simulink model "IEEE123bus_v2019b_Phasor_DPL_ZIPload"  (R2019b)
(part 2 of 12)

  54-55 1 : powerlib/Elements/Distributed Parameters Line  Phases=3  Frequency=60  Resistance=R_1  Inductance=L_1  Capacitance=C_1  Length=275*ft2km  x1=[438.133979265469 4196.77368982038 4204.09231927321;376.991118430775 376.991118430775 376.991118430775;1.68907178229158 -2.40712758914085 2.30524752746821]  x2=[438.133982703911 4196.77368424004 4204.09238504697;376.991118430775 376.991118430775 376.991118430775;1.68907225438477 -2.40712762517757 2.30524750308445]  x3=[0.57767960711374 15.661337452475 12.3899368514742;376.991118430775 376.991118430775 376.991118430775;1.69020592810727 -2.4073134537239 2.30498818329341]  x4=[0.574053544355369 15.6695231741292 12.3933369767456;376.991118430775 376.991118430775 376.991118430775;1.68780051280511 -2.40704970753644 2.30539938237483]  x5=3.44891242524002e-07  V1=ones(3,3)  V2=ones(3,3)  I1=ones(3,3)  I2=ones(3,3)  nHarmo=1  Measurements=None
      settings: SourceProductName=Simscape Electrical
  54-57 3 : powerlib/Elements/Distributed Parameters Line  Phases=3  Frequency=60  Resistance=R_3  Inductance=L_3  Capacitance=C_3  Length=350*ft2km  x1=[442.148345522071 4196.71640972957 4204.09408929467;376.991118430775 376.991118430775 376.991118430775;-0.415145669536993 0.209794158961751 1.78266979920928]  x2=[442.443441248541 4205.29068825861 4210.86387558391;376.991118430775 376.991118430775 376.991118430775;-0.41559689824482 0.208885412947149 1.78176090411138]  x3=[2.56674775762388 185.771024626491 185.574933274428;376.991118430775 376.991118430775 376.991118430775;-1.9761686452555 -1.30181532404798 0.286194361532175]  x4=[2.80709832831061 185.943793008895 185.884239198519;376.991118430775 376.991118430775 376.991118430775;0.738398999629426 1.70643542841195 -3.02471127566214]  x5=4.38952490485094e-07  V1=ones(3,3)  V2=ones(3,3)  I1=ones(3,3)  I2=ones(3,3)  nHarmo=1  Measurements=None
      settings: SourceProductName=Simscape Electrical
  55 : powerlib/Measurements/Three-Phase V-I Measurement  VoltageMeasurement=phase-to-ground  SetLabelV=on  LabelV=V55  Vpu=off  VpuLL=off  CurrentMeasurement=no  SetLabelI=on  LabelI=I65  Ipu=off  Pbase=100e6  Vbase=24900  OutputType=Complex  PhasorSimulation=on  PSBequivalent=0
      settings: SourceProductName=Simscape Electrical
  55 Y Z : Subsystem  mask(Single Phase ZIP Load){Vnom=1.0*2401.78, fnom=60, Pnom=20e3*a, Qnom=10e3*a, LoadType=Constant Z, Vlim=0.7}
      mask prompts: Vnom "Nominal Voltage Vn (Vrms)"; fnom "Nominal Frequency fn (Hz)"; Pnom "Nominal Active power (W)"; Qnom "Nominal Reactive power (VAR)"; LoadType "Load Type"; Vlim "Minimum voltage (pu)"
      mask help:
      | Notes:
      | Single Phase ZIP load model which gets converted to constant Z type if the voltage becomes lower than the Minimum Voltage.
      mask TypeOptions LoadType: Constant Z | constant I | constant P
      mask DialogControl ParameterTabVar0 Prompt: Parameters
      mask DialogControl ParameterTabVar1 Prompt: Type
      mask Display:
      | color('red');
      | A=[-210,-180,-170,-160,-147,-140,-130,-120,-110,-80,-50,-49,-45,-39,-33,-26,-21,-18,-17,-19,-22,-22,-26,-27,-25,-22,-16,-9,-3,2,6,6,4,1,1,-3,-4,-2,2,7,14,20,26,29,30,28,24,24,21,20,21,25,31,37,44,49,50,50,80];
      | B=[-41.5,-41.5,-63,-20,-63,-20,-63,-20,-41.5,-41.5,-41.5,-34,-26,-21,-20,-22,-28,-37,-47,-57,-63,-63,-54,-44,-34,-26,-21,-20,-22,-28,-37,-47,-57,-63,-63,-54,-44,-34,-26,-21,-20,-22,-28,-37,-47,-57,-63,-63,-54,-44,-34,-26,-21,-20,-22,-28,-37,-41.50,-41.5];
      | plot(A,B);
      | color('black');
      | port_label('LConn', 1, '+')
  55-56 1 : powerlib/Elements/Distributed Parameters Line  Phases=3  Frequency=60  Resistance=R_1  Inductance=L_1  Capacitance=C_1  Length=275*ft2km  x1=[438.133982703911 4196.77368424004 4204.09238504697;376.991118430775 376.991118430775 376.991118430775;1.68907225438477 -2.40712762517757 2.30524750308445]  x2=[438.134165148188 4196.77369074888 4204.09236912075;376.991118430775 376.991118430775 376.991118430775;1.68907249725304 -2.4071276498981 2.30524750155646]  x3=[0.577431411639377 15.6627739559426 12.3913283618648;376.991118430775 376.991118430775 376.991118430775;1.68689993805843 -2.40728955810454 2.30521819631482]  x4=[0.574303722649217 15.6680865843111 12.391945096847;376.991118430775 376.991118430775 376.991118430775;1.69112626810043 -2.40707363161943 2.30516940106888]  x5=3.44891242524002e-07  V1=ones(3,3)  V2=ones(3,3)  I1=ones(3,3)  I2=ones(3,3)  nHarmo=1  Measurements=None
      settings: SourceProductName=Simscape Electrical
  56 : powerlib/Measurements/Three-Phase V-I Measurement  VoltageMeasurement=phase-to-ground  SetLabelV=on  LabelV=V56  Vpu=off  VpuLL=off  CurrentMeasurement=no  SetLabelI=on  LabelI=I65  Ipu=off  Pbase=100e6  Vbase=24900  OutputType=Complex  PhasorSimulation=on  PSBequivalent=0
      settings: SourceProductName=Simscape Electrical
  56 Y PQ : Subsystem  mask(Single Phase ZIP Load){Vnom=1.0*2401.78, fnom=60, Pnom=20e3*a, Qnom=10e3*a, LoadType=constant P, Vlim=0.7}
      mask prompts: Vnom "Nominal Voltage Vn (Vrms)"; fnom "Nominal Frequency fn (Hz)"; Pnom "Nominal Active power (W)"; Qnom "Nominal Reactive power (VAR)"; LoadType "Load Type"; Vlim "Minimum voltage (pu)"
      mask help:
      | Notes:
      | Single Phase ZIP load model which gets converted to constant Z type if the voltage becomes lower than the Minimum Voltage.
      mask TypeOptions LoadType: Constant Z | constant I | constant P
      mask DialogControl ParameterTabVar0 Prompt: Parameters
      mask DialogControl ParameterTabVar1 Prompt: Type
      mask Display:
      | color('red');
      | A=[-210,-180,-170,-160,-147,-140,-130,-120,-110,-80,-50,-49,-45,-39,-33,-26,-21,-18,-17,-19,-22,-22,-26,-27,-25,-22,-16,-9,-3,2,6,6,4,1,1,-3,-4,-2,2,7,14,20,26,29,30,28,24,24,21,20,21,25,31,37,44,49,50,50,80];
      | B=[-41.5,-41.5,-63,-20,-63,-20,-63,-20,-41.5,-41.5,-41.5,-34,-26,-21,-20,-22,-28,-37,-47,-57,-63,-63,-54,-44,-34,-26,-21,-20,-22,-28,-37,-47,-57,-63,-63,-54,-44,-34,-26,-21,-20,-22,-28,-37,-47,-57,-63,-63,-54,-44,-34,-26,-21,-20,-22,-28,-37,-41.50,-41.5];
      | plot(A,B);
      | color('black');
      | port_label('LConn', 1, '+')
  57 : powerlib/Measurements/Three-Phase V-I Measurement  VoltageMeasurement=phase-to-ground  SetLabelV=on  LabelV=V57  Vpu=off  VpuLL=off  CurrentMeasurement=no  SetLabelI=on  LabelI=I65  Ipu=off  Pbase=100e6  Vbase=24900  OutputType=Complex  PhasorSimulation=on  PSBequivalent=0
      settings: SourceProductName=Simscape Electrical
  57-58 10 : powerlib/Elements/Distributed Parameters Line  Phases=1  Frequency=60  Resistance=R_10(2,2)  Inductance=L_10(2,2)  Capacitance=C_10(2,2)  Length=250*ft2km  x1=[3435.43252192825;376.991118430775;-2.0999098236995]  x2=[3435.43292902942;376.991118430775;-2.09990968882398]  x3=[6.29780376901278;376.991118430775;-2.09990516681349]  x4=[6.28406360517737;376.991118430775;-2.100031331049]  x5=3.09938851618982e-07  V1=[2.049e+04;377;-2.115]  V2=[2.048e+04;377;-2.115]  I1=[33.62;377;-2.106]  I2=[35.2;377;-2.126]  nHarmo=1  Measurements=None
      settings: SourceProductName=Simscape Electrical
  57-60 3 : powerlib/Elements/Distributed Parameters Line  Phases=3  Frequency=60  Resistance=R_3  Inductance=L_3  Capacitance=C_3  Length=750*ft2km  x1=[442.443441248541 4205.29068825861 4210.86387558391;376.991118430775 376.991118430775 376.991118430775;-0.415786019605193 0.20872918428044 1.78160399294376]  x2=[443.077137686739 4223.67526780051 4225.38226709269;376.991118430775 376.991118430775 376.991118430775;-0.416751865838829 0.206794419050763 1.77966624251521]  x3=[2.57085014444712 185.772514480957 185.583387037946;376.991118430775 376.991118430775 376.991118430775;-1.97623221125093 -1.30182578459823 0.286182634176113]  x4=[2.81031115790824 185.910223378036 185.848218088083;376.991118430775 376.991118430775 376.991118430775;0.738408797497777 1.70599063264223 -3.02515609310221]  x5=9.40612479610915e-07  V1=ones(3,3)  V2=ones(3,3)  I1=ones(3,3)  I2=ones(3,3)  nHarmo=1  Measurements=None
      settings: SourceProductName=Simscape Electrical
  58 : Subsystem
  58 Y I : Subsystem  mask(Single Phase ZIP Load){Vnom=1.0*2401.78, fnom=60, Pnom=20e3*a, Qnom=10e3*a, LoadType=constant I, Vlim=0.7}
      mask prompts: Vnom "Nominal Voltage Vn (Vrms)"; fnom "Nominal Frequency fn (Hz)"; Pnom "Nominal Active power (W)"; Qnom "Nominal Reactive power (VAR)"; LoadType "Load Type"; Vlim "Minimum voltage (pu)"
      mask help:
      | Notes:
      | Single Phase ZIP load model which gets converted to constant Z type if the voltage becomes lower than the Minimum Voltage.
      mask TypeOptions LoadType: Constant Z | constant I | constant P
      mask DialogControl ParameterTabVar0 Prompt: Parameters
      mask DialogControl ParameterTabVar1 Prompt: Type
      mask Display:
      | color('red');
      | A=[-210,-180,-170,-160,-147,-140,-130,-120,-110,-80,-50,-49,-45,-39,-33,-26,-21,-18,-17,-19,-22,-22,-26,-27,-25,-22,-16,-9,-3,2,6,6,4,1,1,-3,-4,-2,2,7,14,20,26,29,30,28,24,24,21,20,21,25,31,37,44,49,50,50,80];
      | B=[-41.5,-41.5,-63,-20,-63,-20,-63,-20,-41.5,-41.5,-41.5,-34,-26,-21,-20,-22,-28,-37,-47,-57,-63,-63,-54,-44,-34,-26,-21,-20,-22,-28,-37,-47,-57,-63,-63,-54,-44,-34,-26,-21,-20,-22,-28,-37,-47,-57,-63,-63,-54,-44,-34,-26,-21,-20,-22,-28,-37,-41.50,-41.5];
      | plot(A,B);
      | color('black');
      | port_label('LConn', 1, '+')
  58-59 10 : powerlib/Elements/Distributed Parameters Line  Phases=1  Frequency=60  Resistance=R_10(2,2)  Inductance=L_10(2,2)  Capacitance=C_10(2,2)  Length=10*ft2km  x1=[3435.43251331732;376.991118430775;-2.09979765583582]  x2=[3435.43252192825;376.991118430775;-2.09979765327296]  x3=[6.29489077198716;376.991118430775;-2.09979765558234]  x4=[6.28801994262156;376.991118430775;-2.09980232984339]  x5=1.23975540647593e-08  V1=[2.049e+04;377;-2.115]  V2=[2.048e+04;377;-2.115]  I1=[33.62;377;-2.106]  I2=[35.2;377;-2.126]  nHarmo=1  Measurements=None
      settings: SourceProductName=Simscape Electrical
  59 : Subsystem
  59 Y PQ : Subsystem  mask(Single Phase ZIP Load){Vnom=1.0*2401.78, fnom=60, Pnom=20e3*a, Qnom=10e3*a, LoadType=constant P, Vlim=0.7}
      mask prompts: Vnom "Nominal Voltage Vn (Vrms)"; fnom "Nominal Frequency fn (Hz)"; Pnom "Nominal Active power (W)"; Qnom "Nominal Reactive power (VAR)"; LoadType "Load Type"; Vlim "Minimum voltage (pu)"
      mask help:
      | Notes:
      | Single Phase ZIP load model which gets converted to constant Z type if the voltage becomes lower than the Minimum Voltage.
      mask TypeOptions LoadType: Constant Z | constant I | constant P
      mask DialogControl ParameterTabVar0 Prompt: Parameters
      mask DialogControl ParameterTabVar1 Prompt: Type
      mask Display:
      | color('red');
      | A=[-210,-180,-170,-160,-147,-140,-130,-120,-110,-80,-50,-49,-45,-39,-33,-26,-21,-18,-17,-19,-22,-22,-26,-27,-25,-22,-16,-9,-3,2,6,6,4,1,1,-3,-4,-2,2,7,14,20,26,29,30,28,24,24,21,20,21,25,31,37,44,49,50,50,80];
      | B=[-41.5,-41.5,-63,-20,-63,-20,-63,-20,-41.5,-41.5,-41.5,-34,-26,-21,-20,-22,-28,-37,-47,-57,-63,-63,-54,-44,-34,-26,-21,-20,-22,-28,-37,-47,-57,-63,-63,-54,-44,-34,-26,-21,-20,-22,-28,-37,-47,-57,-63,-63,-54,-44,-34,-26,-21,-20,-22,-28,-37,-41.50,-41.5];
      | plot(A,B);
      | color('black');
      | port_label('LConn', 1, '+')
  59-94 : powerlib/Elements/Breaker  InitialState=0  SwitchingTimes="[1/60  5/60]"  External=off  BreakerResistance=0.01  SnubberResistance=1e6  SnubberCapacitance=inf  Measurements=None  MoreParameters=on  NoBreakLoop=off
      settings: SourceProductName=Simscape Electrical
  6 : Subsystem
  6 Y Z : Subsystem  mask(Single Phase ZIP Load){Vnom=1.0*2401.78, fnom=60, Pnom=40e3*a, Qnom=20e3*a, LoadType=Constant Z, Vlim=0.7}
      mask prompts: Vnom "Nominal Voltage Vn (Vrms)"; fnom "Nominal Frequency fn (Hz)"; Pnom "Nominal Active power (W)"; Qnom "Nominal Reactive power (VAR)"; LoadType "Load Type"; Vlim "Minimum voltage (pu)"
      mask help:
      | Notes:
      | Single Phase ZIP load model which gets converted to constant Z type if the voltage becomes lower than the Minimum Voltage.
      mask TypeOptions LoadType: Constant Z | constant I | constant P
      mask DialogControl ParameterTabVar0 Prompt: Parameters
      mask DialogControl ParameterTabVar1 Prompt: Type
      mask Display:
      | color('red');
      | A=[-210,-180,-170,-160,-147,-140,-130,-120,-110,-80,-50,-49,-45,-39,-33,-26,-21,-18,-17,-19,-22,-22,-26,-27,-25,-22,-16,-9,-3,2,6,6,4,1,1,-3,-4,-2,2,7,14,20,26,29,30,28,24,24,21,20,21,25,31,37,44,49,50,50,80];
      | B=[-41.5,-41.5,-63,-20,-63,-20,-63,-20,-41.5,-41.5,-41.5,-34,-26,-21,-20,-22,-28,-37,-47,-57,-63,-63,-54,-44,-34,-26,-21,-20,-22,-28,-37,-47,-57,-63,-63,-54,-44,-34,-26,-21,-20,-22,-28,-37,-47,-57,-63,-63,-54,-44,-34,-26,-21,-20,-22,-28,-37,-41.50,-41.5];
      | plot(A,B);
      | color('black');
      | port_label('LConn', 1, '+')
  60 : powerlib/Measurements/Three-Phase V-I Measurement  VoltageMeasurement=phase-to-ground  SetLabelV=on  LabelV=V60  Vpu=off  VpuLL=off  CurrentMeasurement=no  SetLabelI=on  LabelI=I65  Ipu=off  Pbase=100e6  Vbase=24900  OutputType=Complex  PhasorSimulation=on  PSBequivalent=0
      settings: SourceProductName=Simscape Electrical
  60 Y PQ : Subsystem  mask(Single Phase ZIP Load){Vnom=1.0*2401.78, fnom=60, Pnom=20e3*a, Qnom=10e3*a, LoadType=constant P, Vlim=0.7}
      mask prompts: Vnom "Nominal Voltage Vn (Vrms)"; fnom "Nominal Frequency fn (Hz)"; Pnom "Nominal Active power (W)"; Qnom "Nominal Reactive power (VAR)"; LoadType "Load Type"; Vlim "Minimum voltage (pu)"
      mask help:
      | Notes:
      | Single Phase ZIP load model which gets converted to constant Z type if the voltage becomes lower than the Minimum Voltage.
      mask TypeOptions LoadType: Constant Z | constant I | constant P
      mask DialogControl ParameterTabVar0 Prompt: Parameters
      mask DialogControl ParameterTabVar1 Prompt: Type
      mask Display:
      | color('red');
      | A=[-210,-180,-170,-160,-147,-140,-130,-120,-110,-80,-50,-49,-45,-39,-33,-26,-21,-18,-17,-19,-22,-22,-26,-27,-25,-22,-16,-9,-3,2,6,6,4,1,1,-3,-4,-2,2,7,14,20,26,29,30,28,24,24,21,20,21,25,31,37,44,49,50,50,80];
      | B=[-41.5,-41.5,-63,-20,-63,-20,-63,-20,-41.5,-41.5,-41.5,-34,-26,-21,-20,-22,-28,-37,-47,-57,-63,-63,-54,-44,-34,-26,-21,-20,-22,-28,-37,-47,-57,-63,-63,-54,-44,-34,-26,-21,-20,-22,-28,-37,-47,-57,-63,-63,-54,-44,-34,-26,-21,-20,-22,-28,-37,-41.50,-41.5];
      | plot(A,B);
      | color('black');
      | port_label('LConn', 1, '+')
  60-1 : powerlib/Elements/Three-Phase Breaker  InitialState=closed  SwitchA=off  SwitchB=off  SwitchC=off  SwitchTimes="[1/60  5/60]"  External=off  BreakerResistance=1e-6  SnubberResistance=1e6  SnubberCapacitance=inf  Measurements=None
      settings: SourceProductName=Simscape Electrical
  60-61 5 : powerlib/Elements/Distributed Parameters Line  Phases=3  Frequency=60  Resistance=R_5  Inductance=L_5  Capacitance=C_5  Length=550*ft2km  x1=[444.012645413385 4225.42266060109 4223.62125047857;376.991118430775 376.991118430775 376.991118430775;2.49497234010463 0.298404870388615 1.87127772270801]  x2=[444.012528550903 4225.41947596016 4223.61751082761;376.991118430775 376.991118430775 376.991118430775;2.49497212075308 0.298404632695918 1.87127735759577]  x3=[0.582941938221517 15.7350722313925 12.412214405866;376.991118430775 376.991118430775 376.991118430775;2.49542314249947 0.300513509954508 1.8740159956356]  x4=[0.584198142948021 15.8083228008512 12.4853955100635;376.991118430775 376.991118430775 376.991118430775;2.49426251890333 0.296090505039898 1.86834094582853]  x5=6.89782485048005e-07  V1=ones(3,3)  V2=ones(3,3)  I1=ones(3,3)  I2=ones(3,3)  nHarmo=1  Measurements=None
      settings: SourceProductName=Simscape Electrical
  60-62 12 : powerlib/Elements/Distributed Parameters Line  Phases=3  Frequency=60  Resistance=R_12  Inductance=L_12  Capacitance=C_12  Length=250*ft2km  x1=[55.9080637748695 4230.58957773142 4221.53713212597;376.991118430775 376.991118430775 376.991118430775;-2.11125455967542 -0.531784886489894 -2.10256121564759]  x2=[55.9081119023914 4230.59053489679 4221.53785585336;376.991118430775 376.991118430775 376.991118430775;-2.11125220052181 -0.531785854790702 -2.10256215821121]  x3=[0.409811763631933 47.322508785806 52.7495421781275;376.991118430775 376.991118430775 376.991118430775;-2.10971013269117 -0.533494472470248 -2.10413818670958]  x4=[0.408303432755578 47.3605643476315 52.7847250961121;376.991118430775 376.991118430775 376.991118430775;-2.11323797588244 -0.530361891184764 -2.1012407263576]  x5=1.15320558205325e-06  V1=ones(3,3)  V2=ones(3,3)  I1=ones(3,3)  I2=ones(3,3)  nHarmo=1  Measurements=None
      settings: SourceProductName=Simscape Electrical
  61 : powerlib/Measurements/Three-Phase V-I Measurement  VoltageMeasurement=phase-to-ground  SetLabelV=on  LabelV=V61  Vpu=off  VpuLL=off  CurrentMeasurement=no  SetLabelI=on  LabelI=I65  Ipu=off  Pbase=100e6  Vbase=24900  OutputType=Complex  PhasorSimulation=on  PSBequivalent=0
      settings: SourceProductName=Simscape Electrical
  61-610 : powerlib/Elements/Three-Phase Breaker  InitialState=closed  SwitchA=off  SwitchB=off  SwitchC=off  SwitchTimes="[1/60  5/60]"  External=off  BreakerResistance=1e-6  SnubberResistance=1e6  SnubberCapacitance=inf  Measurements=None
      settings: SourceProductName=Simscape Electrical
  610 : powerlib/Measurements/Three-Phase V-I Measurement  VoltageMeasurement=phase-to-phase  SetLabelV=on  LabelV=V610  Vpu=off  VpuLL=off  CurrentMeasurement=no  SetLabelI=on  LabelI=I65  Ipu=off  Pbase=100e6  Vbase=24900  OutputType=Complex  PhasorSimulation=on  PSBequivalent=0
      settings: SourceProductName=Simscape Electrical
  62 : powerlib/Measurements/Three-Phase V-I Measurement  VoltageMeasurement=phase-to-ground  SetLabelV=on  LabelV=V62  Vpu=off  VpuLL=off  CurrentMeasurement=no  SetLabelI=on  LabelI=I65  Ipu=off  Pbase=100e6  Vbase=24900  OutputType=Complex  PhasorSimulation=on  PSBequivalent=0
      settings: SourceProductName=Simscape Electrical
  62 Y Z : Subsystem  mask(Single Phase ZIP Load){Vnom=1.0*2401.78, fnom=60, Pnom=40e3*a, Qnom=20e3*a, LoadType=Constant Z, Vlim=0.7}
      mask prompts: Vnom "Nominal Voltage Vn (Vrms)"; fnom "Nominal Frequency fn (Hz)"; Pnom "Nominal Active power (W)"; Qnom "Nominal Reactive power (VAR)"; LoadType "Load Type"; Vlim "Minimum voltage (pu)"
      mask help:
      | Notes:
      | Single Phase ZIP load model which gets converted to constant Z type if the voltage becomes lower than the Minimum Voltage.
      mask TypeOptions LoadType: Constant Z | constant I | constant P
      mask DialogControl ParameterTabVar0 Prompt: Parameters
      mask DialogControl ParameterTabVar1 Prompt: Type
      mask Display:
      | color('red');
      | A=[-210,-180,-170,-160,-147,-140,-130,-120,-110,-80,-50,-49,-45,-39,-33,-26,-21,-18,-17,-19,-22,-22,-26,-27,-25,-22,-16,-9,-3,2,6,6,4,1,1,-3,-4,-2,2,7,14,20,26,29,30,28,24,24,21,20,21,25,31,37,44,49,50,50,80];
      | B=[-41.5,-41.5,-63,-20,-63,-20,-63,-20,-41.5,-41.5,-41.5,-34,-26,-21,-20,-22,-28,-37,-47,-57,-63,-63,-54,-44,-34,-26,-21,-20,-22,-28,-37,-47,-57,-63,-63,-54,-44,-34,-26,-21,-20,-22,-28,-37,-47,-57,-63,-63,-54,-44,-34,-26,-21,-20,-22,-28,-37,-41.50,-41.5];
      | plot(A,B);
      | color('black');
      | port_label('LConn', 1, '+')
  62-63 12 : powerlib/Elements/Distributed Parameters Line  Phases=3  Frequency=60  Resistance=R_12  Inductance=L_12  Capacitance=C_12  Length=175*ft2km  x1=[55.9081119023914 4230.59053489679 4221.53785585336;376.991118430775 376.991118430775 376.991118430775;-2.11112177604316 -0.53170055742354 -2.10248579753503]  x2=[55.908128877514 4230.59109519292 4221.5382057241;376.991118430775 376.991118430775 376.991118430775;-2.11112321460848 -0.53170114392752 -2.10248635550861]  x3=[0.408923617366455 47.3304210988168 52.7572720335478;376.991118430775 376.991118430775 376.991118430775;-2.11334381642661 -0.53315126804625 -2.10378447749276]  x4=[0.409355021574173 47.3642530596418 52.7910307638753;376.991118430775 376.991118430775 376.991118430775;-2.10920772556812 -0.530450444417656 -2.10136664224366]  x5=8.07243907437275e-07  V1=ones(3,3)  V2=ones(3,3)  I1=ones(3,3)  I2=ones(3,3)  nHarmo=1  Measurements=None
      settings: SourceProductName=Simscape Electrical
  63 : powerlib/Measurements/Three-Phase V-I Measurement  VoltageMeasurement=phase-to-ground  SetLabelV=on  LabelV=V63  Vpu=off  VpuLL=off  CurrentMeasurement=no  SetLabelI=on  LabelI=I65  Ipu=off  Pbase=100e6  Vbase=24900  OutputType=Complex  PhasorSimulation=on  PSBequivalent=0
      settings: SourceProductName=Simscape Electrical
  63 Y PQ : Subsystem  mask(Single Phase ZIP Load){Vnom=1.0*2401.78, fnom=60, Pnom=40e3*a, Qnom=20e3*a, LoadType=constant P, Vlim=0.7}
      mask prompts: Vnom "Nominal Voltage Vn (Vrms)"; fnom "Nominal Frequency fn (Hz)"; Pnom "Nominal Active power (W)"; Qnom "Nominal Reactive power (VAR)"; LoadType "Load Type"; Vlim "Minimum voltage (pu)"
      mask help:
      | Notes:
      | Single Phase ZIP load model which gets converted to constant Z type if the voltage becomes lower than the Minimum Voltage.
      mask TypeOptions LoadType: Constant Z | constant I | constant P
      mask DialogControl ParameterTabVar0 Prompt: Parameters
      mask DialogControl ParameterTabVar1 Prompt: Type
      mask Display:
      | color('red');
      | A=[-210,-180,-170,-160,-147,-140,-130,-120,-110,-80,-50,-49,-45,-39,-33,-26,-21,-18,-17,-19,-22,-22,-26,-27,-25,-22,-16,-9,-3,2,6,6,4,1,1,-3,-4,-2,2,7,14,20,26,29,30,28,24,24,21,20,21,25,31,37,44,49,50,50,80];
      | B=[-41.5,-41.5,-63,-20,-63,-20,-63,-20,-41.5,-41.5,-41.5,-34,-26,-21,-20,-22,-28,-37,-47,-57,-63,-63,-54,-44,-34,-26,-21,-20,-22,-28,-37,-47,-57,-63,-63,-54,-44,-34,-26,-21,-20,-22,-28,-37,-47,-57,-63,-63,-54,-44,-34,-26,-21,-20,-22,-28,-37,-41.50,-41.5];
      | plot(A,B);
      | color('black');
      | port_label('LConn', 1, '+')
  63-64 12 : powerlib/Elements/Distributed Parameters Line  Phases=3  Frequency=60  Resistance=R_12  Inductance=L_12  Capacitance=C_12  Length=350*ft2km  x1=[55.908128877514 4230.59109519292 4221.5382057241;376.991118430775 376.991118430775 376.991118430775;-2.111427538392 -0.531900171117565 -2.10266453041969]  x2=[55.9078369500797 4230.5918139492 4221.5385862525;376.991118430775 376.991118430775 376.991118430775;-2.11142619644169 -0.531901078867907 -2.10266543956144]  x3=[0.407735051336149 47.3189818762066 52.7415879960659;376.991118430775 376.991118430775 376.991118430775;-2.10917596383347 -0.533126104122833 -2.10380861674724]  x4=[0.410163400855526 47.3485738498202 52.773902727855;376.991118430775 376.991118430775 376.991118430775;-2.11427147796887 -0.53107391768484 -2.10187836803492]  x5=1.61448781487455e-06  V1=ones(3,3)  V2=ones(3,3)  I1=ones(3,3)  I2=ones(3,3)  nHarmo=1  Measurements=None
      settings: SourceProductName=Simscape Electrical
  64 : powerlib/Measurements/Three-Phase V-I Measurement  VoltageMeasurement=phase-to-ground  SetLabelV=on  LabelV=V64  Vpu=off  VpuLL=off  CurrentMeasurement=no  SetLabelI=on  LabelI=I65  Ipu=off  Pbase=100e6  Vbase=24900  OutputType=Complex  PhasorSimulation=on  PSBequivalent=0
      settings: SourceProductName=Simscape Electrical
  64 Y I : Subsystem  mask(Single Phase ZIP Load){Vnom=1.0*2401.78, fnom=60, Pnom=75e3*a, Qnom=35e3*a, LoadType=constant I, Vlim=0.7}
      mask prompts: Vnom "Nominal Voltage Vn (Vrms)"; fnom "Nominal Frequency fn (Hz)"; Pnom "Nominal Active power (W)"; Qnom "Nominal Reactive power (VAR)"; LoadType "Load Type"; Vlim "Minimum voltage (pu)"
      mask help:
      | Notes:
      | Single Phase ZIP load model which gets converted to constant Z type if the voltage becomes lower than the Minimum Voltage.
      mask TypeOptions LoadType: Constant Z | constant I | constant P
      mask DialogControl ParameterTabVar0 Prompt: Parameters
      mask DialogControl ParameterTabVar1 Prompt: Type
      mask Display:
      | color('red');
      | A=[-210,-180,-170,-160,-147,-140,-130,-120,-110,-80,-50,-49,-45,-39,-33,-26,-21,-18,-17,-19,-22,-22,-26,-27,-25,-22,-16,-9,-3,2,6,6,4,1,1,-3,-4,-2,2,7,14,20,26,29,30,28,24,24,21,20,21,25,31,37,44,49,50,50,80];
      | B=[-41.5,-41.5,-63,-20,-63,-20,-63,-20,-41.5,-41.5,-41.5,-34,-26,-21,-20,-22,-28,-37,-47,-57,-63,-63,-54,-44,-34,-26,-21,-20,-22,-28,-37,-47,-57,-63,-63,-54,-44,-34,-26,-21,-20,-22,-28,-37,-47,-57,-63,-63,-54,-44,-34,-26,-21,-20,-22,-28,-37,-41.50,-41.5];
      | plot(A,B);
      | color('black');
      | port_label('LConn', 1, '+')
  64-65 12 : powerlib/Elements/Distributed Parameters Line  Phases=3  Frequency=60  Resistance=R_12  Inductance=L_12  Capacitance=C_12  Length=425*ft2km  x1=[55.9078369500797 4230.5918139492 4221.5385862525;376.991118430775 376.991118430775 376.991118430775;-2.11155662092034 -0.531986376235069 -2.10274180023762]  x2=[55.9078682558492 4230.59178555001 4221.53855219661;376.991118430775 376.991118430775 376.991118430775;-2.11155025867436 -0.53198707006632 -2.10274248430972]  x3=[0.4096774495443 47.3131665016492 52.7373394629299;376.991118430775 376.991118430775 376.991118430775;-2.10866668592754 -0.532814088725115 -2.10352935181206]  x4=[0.408058398109022 47.3427535827325 52.7640731119049;376.991118430775 376.991118430775 376.991118430775;-2.11519246354483 -0.531643187308702 -2.10238804129711]  x5=1.96044948949052e-06  V1=ones(3,3)  V2=ones(3,3)  I1=ones(3,3)  I2=ones(3,3)  nHarmo=1  Measurements=None
      settings: SourceProductName=Simscape Electrical
  65 : powerlib/Measurements/Three-Phase V-I Measurement  VoltageMeasurement=phase-to-ground  SetLabelV=on  LabelV=V65  Vpu=off  VpuLL=off  CurrentMeasurement=yes  SetLabelI=on  LabelI=I65  Ipu=off  Pbase=100e6  Vbase=24900  OutputType=Complex  PhasorSimulation=on  PSBequivalent=0
      settings: SourceProductName=Simscape Electrical
  65 D Z : Subsystem  mask(Three Phase Delta ZIP Load (Phasor)){Vnom=4160, fnom=60, Pnom=[35 35 70]*1e3*a, Qnom=[25 25 50]*1e3*a, LoadType=Constant Z, Vlim=0.7}
      mask prompts: Vnom "Nominal Ph-Ph Voltage (Vrms)"; fnom "Nominal Frequency fn (Hz)"; Pnom "Nominal Per Phase Active Power [Pab Pbc Pca] (W)"; Qnom "Nominal Per Phase Reactive Power [Qab Qbc Qca] (VAR)"; LoadType "Load Type"; Vlim "Minimum Voltage (pu)"
      mask help:
      | Notes:
      | Three Phase Delta Connected ZIP load model which gets converted to constant Z type if the voltage becomes lower than the Minimum Voltage.
      mask TypeOptions LoadType: Constant Z | Constant I | Constant P
      mask DialogControl ParameterTabVar0 Prompt: Parameters
      mask DialogControl ParameterTabVar01 Prompt: Type
      mask Display:
      | color('red');
      | %load figure 0deg
      | A=[-210,-180,-170,-160,-147,-140,-130,-120,-110,-80,-50,-49,-45,-39,-33,-26,-21,-18,-17,-19,-22,-22,-26,-27,-25,-22,-16,-9,-3,2,6,6,4,1,1,-3,-4,-2,2,7,14,20,26,29,30,28,24,24,21,20,21,25,31,37,44,49,50,50,80];
      | B=[-41.5,-41.5,-63,-20,-63,-20,-63,-20,-41.5,-41.5,-41.5,-34,-26,-21,-20,-22,-28,-37,-47,-57,-63,-63,-54,-44,-34,-26,-21,-20,-22,-28,-37,-47,-57,-63,-63,-54,-44,-34,-26,-21,-20,-22,-28,-37,-47,-57,-63,-63,-54,-44,-34,-26,-21,-20,-22,-28,-37,-41.50,-41.5];
      | plot(A,B);
      | 
      | %load figure 0deg inverted
      | A1=[-80,-50,-49,-45,-39,-33,-26,-21,-18,-17,-19,-22,-22,-26,-27,-25,-22,-16,-9,-3,2,6,6,4,1,1,-3,-4,-2,2,7,14,20,26,29,30,28,24,24,21,20,21,25,31,37,44,49,50,50,80,110,120,130,143,150,160,170,180,210];
      | B1=[-41.5,-41.5,-34,-26,-21,-20,-22,-28,-37,-47,-57,-63,-63,-54,-44,-34,-26,-21,-20,-22,-28,-37,-47,-57,-63,-63,-54,-44,-34,-26,-21,-20,-22,-28,-37,-47,-57,-63,-63,-54,-44,-34,-26,-21,-20,-22,-28,-37,-41.5,-41.5,-41.5,-63,-20,-63,-20,-63,-20,-41.5,-41.5];
      | 
      | 
      | %load figure -120deg
      | c=1*exp(sqrt(-1)*(-60*pi/180));
      | l=A1+j*B1;
      | m=l*c;
      | E=real(m);F=imag(m);
      | E=E+10.94;F=F+161.1;
      | plot(E,F);
      | 
      | %load figure +120deg
      | c=1*exp(sqrt(-1)*(60*pi/180));
      | l=A1+j*B1;
      | m=l*c;
      | G=real(m);
      | H=imag(m);
      | G=G-205.94;H=H+48.53;
      | plot(G,H);
      | 
      | color('black');
      | port_label('LConn', 1, 'A')
      | port_label('LConn', 2, 'B')
      | port_label('LConn', 3, 'C')
  65-66 12 : powerlib/Elements/Distributed Parameters Line  Phases=3  Frequency=60  Resistance=R_12  Inductance=L_12  Capacitance=C_12  Length=325*ft2km  x1=[55.9078682558492 4230.59178555001 4221.53855219661;376.991118430775 376.991118430775 376.991118430775;-2.1113763593695 -0.531873340243438 -2.10264067007481]  x2=[55.9078965570197 4230.59190041181 4221.53877217118;376.991118430775 376.991118430775 376.991118430775;-2.11137052111276 -0.531873469510167 -2.10264081999727]  x3=[0.409946953161696 47.3335790646025 52.7593520742274;376.991118430775 376.991118430775 376.991118430775;-2.10774697816406 -0.532217327174848 -2.10299518711263]  x4=[0.408007794592192 47.3378070213513 52.7607820462584;376.991118430775 376.991118430775 376.991118430775;-2.11558381639439 -0.531899184200729 -2.10261726800257]  x5=1.49916725666922e-06  V1=ones(3,3)  V2=ones(3,3)  I1=ones(3,3)  I2=ones(3,3)  nHarmo=1  Measurements=None
      settings: SourceProductName=Simscape Electrical
  66 : powerlib/Measurements/Three-Phase V-I Measurement  VoltageMeasurement=phase-to-ground  SetLabelV=on  LabelV=V66  Vpu=off  VpuLL=off  CurrentMeasurement=no  SetLabelI=on  LabelI=I65  Ipu=off  Pbase=100e6  Vbase=24900  OutputType=Complex  PhasorSimulation=on  PSBequivalent=0
      settings: SourceProductName=Simscape Electrical
  66 Y PQ : Subsystem  mask(Single Phase ZIP Load){Vnom=1.0*2401.78, fnom=60, Pnom=75e3*a, Qnom=35e3*a, LoadType=constant P, Vlim=0.7}
      mask prompts: Vnom "Nominal Voltage Vn (Vrms)"; fnom "Nominal Frequency fn (Hz)"; Pnom "Nominal Active power (W)"; Qnom "Nominal Reactive power (VAR)"; LoadType "Load Type"; Vlim "Minimum voltage (pu)"
      mask help:
      | Notes:
      | Single Phase ZIP load model which gets converted to constant Z type if the voltage becomes lower than the Minimum Voltage.
      mask TypeOptions LoadType: Constant Z | constant I | constant P
      mask DialogControl ParameterTabVar0 Prompt: Parameters
      mask DialogControl ParameterTabVar1 Prompt: Type
      mask Display:
      | color('red');
      | A=[-210,-180,-170,-160,-147,-140,-130,-120,-110,-80,-50,-49,-45,-39,-33,-26,-21,-18,-17,-19,-22,-22,-26,-27,-25,-22,-16,-9,-3,2,6,6,4,1,1,-3,-4,-2,2,7,14,20,26,29,30,28,24,24,21,20,21,25,31,37,44,49,50,50,80];
      | B=[-41.5,-41.5,-63,-20,-63,-20,-63,-20,-41.5,-41.5,-41.5,-34,-26,-21,-20,-22,-28,-37,-47,-57,-63,-63,-54,-44,-34,-26,-21,-20,-22,-28,-37,-47,-57,-63,-63,-54,-44,-34,-26,-21,-20,-22,-28,-37,-47,-57,-63,-63,-54,-44,-34,-26,-21,-20,-22,-28,-37,-41.50,-41.5];
      | plot(A,B);
      | color('black');
      | port_label('LConn', 1, '+')
  67 : powerlib/Measurements/Three-Phase V-I Measurement  VoltageMeasurement=phase-to-ground  SetLabelV=on  LabelV=V67  Vpu=off  VpuLL=off  CurrentMeasurement=no  SetLabelI=on  LabelI=I65  Ipu=off  Pbase=100e6  Vbase=24900  OutputType=Complex  PhasorSimulation=on  PSBequivalent=0
      settings: SourceProductName=Simscape Electrical
  67-68 9 : powerlib/Elements/Distributed Parameters Line  Phases=1  Frequency=60  Resistance=R_9(1,1)  Inductance=L_9(1,1)  Capacitance=C_9(1,1)  Length=200*ft2km  x1=[3458.2040924721;376.991118430775;-0.00997406199651134]  x2=[3458.20354338365;376.991118430775;-0.00997430817436671]  x3=[6.31891140278979;376.991118430775;-0.0104776746439766]  x4=[6.34657266029751;376.991118430775;-0.00956616376296402]  x5=2.47951081295186e-07  V1=[2.049e+04;377;-2.115]  V2=[2.048e+04;377;-2.115]  I1=[33.62;377;-2.106]  I2=[35.2;377;-2.126]  nHarmo=1  Measurements=None
      settings: SourceProductName=Simscape Electrical
  67-72 3 : powerlib/Elements/Distributed Parameters Line  Phases=3  Frequency=60  Resistance=R_3  Inductance=L_3  Capacitance=C_3  Length=275*ft2km  x1=[443.372743435122 4232.25892858286 4232.16211596932;376.991118430775 376.991118430775 376.991118430775;-0.416976568435667 0.206083528596057 1.77895345394237]  x2=[443.603864090973 4239.00541261997 4237.49079663196;376.991118430775 376.991118430775 376.991118430775;-0.417326988044593 0.205382268298549 1.77824945384504]  x3=[2.55557537522218 185.752851770927 185.556114030351;376.991118430775 376.991118430775 376.991118430775;-1.97350532867016 -1.30069039397134 0.287263381590106]  x4=[2.79349756184913 185.823460144677 185.738159747128;376.991118430775 376.991118430775 376.991118430775;0.737631593550109 1.70640536238687 -3.02482877829137]  x5=3.44891242524002e-07  V1=ones(3,3)  V2=ones(3,3)  I1=ones(3,3)  I2=ones(3,3)  nHarmo=1  Measurements=None
      settings: SourceProductName=Simscape Electrical
  67-97 3 : powerlib/Elements/Distributed Parameters Line  Phases=3  Frequency=60  Resistance=R_3  Inductance=L_3  Capacitance=C_3  Length=250*ft2km  x1=[443.372743435122 4232.25892858286 4232.16211596932;376.991118430775 376.991118430775 376.991118430775;-0.416964748350644 0.206093292887726 1.77896326089034]  x2=[443.373227084636 4232.2593632206 4232.16270175339;376.991118430775 376.991118430775 376.991118430775;-0.416965831798407 0.206093045516371 1.7789630646897]  x3=[0.580047745954408 12.4529945543642 15.7828273942649;376.991118430775 376.991118430775 376.991118430775;-0.428193151939215 0.20422859869058 1.77698414970922]  x4=[0.585532617715679 12.4964437997908 15.8124131522216;376.991118430775 376.991118430775 376.991118430775;-0.40596025617013 0.207853782520193 1.78084049398028]  x5=3.13537493203638e-07  V1=ones(3,3)  V2=ones(3,3)  I1=ones(3,3)  I2=ones(3,3)  nHarmo=1  Measurements=None
      settings: SourceProductName=Simscape Electrical
  68 : Subsystem
  68 Y PQ : Subsystem  mask(Single Phase ZIP Load){Vnom=1.0*2401.78, fnom=60, Pnom=20e3*a, Qnom=10e3*a, LoadType=constant P, Vlim=0.7}
      mask prompts: Vnom "Nominal Voltage Vn (Vrms)"; fnom "Nominal Frequency fn (Hz)"; Pnom "Nominal Active power (W)"; Qnom "Nominal Reactive power (VAR)"; LoadType "Load Type"; Vlim "Minimum voltage (pu)"
      mask help:
      | Notes:
      | Single Phase ZIP load model which gets converted to constant Z type if the voltage becomes lower than the Minimum Voltage.
      mask TypeOptions LoadType: Constant Z | constant I | constant P
      mask DialogControl ParameterTabVar0 Prompt: Parameters
      mask DialogControl ParameterTabVar1 Prompt: Type
      mask Display:
      | color('red');
      | A=[-210,-180,-170,-160,-147,-140,-130,-120,-110,-80,-50,-49,-45,-39,-33,-26,-21,-18,-17,-19,-22,-22,-26,-27,-25,-22,-16,-9,-3,2,6,6,4,1,1,-3,-4,-2,2,7,14,20,26,29,30,28,24,24,21,20,21,25,31,37,44,49,50,50,80];
      | B=[-41.5,-41.5,-63,-20,-63,-20,-63,-20,-41.5,-41.5,-41.5,-34,-26,-21,-20,-22,-28,-37,-47,-57,-63,-63,-54,-44,-34,-26,-21,-20,-22,-28,-37,-47,-57,-63,-63,-54,-44,-34,-26,-21,-20,-22,-28,-37,-47,-57,-63,-63,-54,-44,-34,-26,-21,-20,-22,-28,-37,-41.50,-41.5];
      | plot(A,B);
      | color('black');
      | port_label('LConn', 1, '+')
  68-69 9 : powerlib/Elements/Distributed Parameters Line  Phases=1  Frequency=60  Resistance=R_9(1,1)  Inductance=L_9(1,1)  Capacitance=C_9(1,1)  Length=275*ft2km  x1=[3458.20354338365;376.991118430775;-0.0100093614326618]  x2=[3458.20297836085;376.991118430775;-0.0100096156875461]  x3=[6.32220303585171;376.991118430775;-0.0104190223540927]  x4=[6.34294999092737;376.991118430775;-0.00972961677725644]  x5=3.4093273678088e-07  V1=[2.049e+04;377;-2.115]  V2=[2.048e+04;377;-2.115]  I1=[33.62;377;-2.106]  I2=[35.2;377;-2.126]  nHarmo=1  Measurements=None
      settings: SourceProductName=Simscape Electrical
  69 : Subsystem
  69 Y PQ : Subsystem  mask(Single Phase ZIP Load){Vnom=1.0*2401.78, fnom=60, Pnom=40e3*a, Qnom=20e3*a, LoadType=constant P, Vlim=0.7}
      mask prompts: Vnom "Nominal Voltage Vn (Vrms)"; fnom "Nominal Frequency fn (Hz)"; Pnom "Nominal Active power (W)"; Qnom "Nominal Reactive power (VAR)"; LoadType "Load Type"; Vlim "Minimum voltage (pu)"
      mask help:
      | Notes:
      | Single Phase ZIP load model which gets converted to constant Z type if the voltage becomes lower than the Minimum Voltage.
      mask TypeOptions LoadType: Constant Z | constant I | constant P
      mask DialogControl ParameterTabVar0 Prompt: Parameters
      mask DialogControl ParameterTabVar1 Prompt: Type
      mask Display:
      | color('red');
      | A=[-210,-180,-170,-160,-147,-140,-130,-120,-110,-80,-50,-49,-45,-39,-33,-26,-21,-18,-17,-19,-22,-22,-26,-27,-25,-22,-16,-9,-3,2,6,6,4,1,1,-3,-4,-2,2,7,14,20,26,29,30,28,24,24,21,20,21,25,31,37,44,49,50,50,80];
      | B=[-41.5,-41.5,-63,-20,-63,-20,-63,-20,-41.5,-41.5,-41.5,-34,-26,-21,-20,-22,-28,-37,-47,-57,-63,-63,-54,-44,-34,-26,-21,-20,-22,-28,-37,-47,-57,-63,-63,-54,-44,-34,-26,-21,-20,-22,-28,-37,-47,-57,-63,-63,-54,-44,-34,-26,-21,-20,-22,-28,-37,-41.50,-41.5];
      | plot(A,B);
      | color('black');
      | port_label('LConn', 1, '+')
  69-70 9 : powerlib/Elements/Distributed Parameters Line  Phases=1  Frequency=60  Resistance=R_9(1,1)  Inductance=L_9(1,1)  Capacitance=C_9(1,1)  Length=325*ft2km  x1=[3458.20297836085;376.991118430775;-0.0100329845264095]  x2=[3458.20251991098;376.991118430775;-0.010033181055214]  x3=[6.32555047487211;376.991118430775;-0.01031375998793]  x4=[6.33938124215797;376.991118430775;-0.00990475538991943]  x5=4.02920507104677e-07  V1=[2.049e+04;377;-2.115]  V2=[2.048e+04;377;-2.115]  I1=[33.62;377;-2.106]  I2=[35.2;377;-2.126]  nHarmo=1  Measurements=None
      settings: SourceProductName=Simscape Electrical
  7 : powerlib/Measurements/Three-Phase V-I Measurement  VoltageMeasurement=phase-to-ground  SetLabelV=on  LabelV=V7  Vpu=off  VpuLL=off  CurrentMeasurement=no  SetLabelI=on  LabelI=I800  Ipu=off  Pbase=100e6  Vbase=24900  OutputType=Complex  PhasorSimulation=on  PSBequivalent=0
      settings: SourceProductName=Simscape Electrical
  7 Y PQ : Subsystem  mask(Single Phase ZIP Load){Vnom=1.0*2401.78, fnom=60, Pnom=20e3*a, Qnom=10e3*a, LoadType=constant P, Vlim=0.7}
      mask prompts: Vnom "Nominal Voltage Vn (Vrms)"; fnom "Nominal Frequency fn (Hz)"; Pnom "Nominal Active power (W)"; Qnom "Nominal Reactive power (VAR)"; LoadType "Load Type"; Vlim "Minimum voltage (pu)"
      mask help:
      | Notes:
      | Single Phase ZIP load model which gets converted to constant Z type if the voltage becomes lower than the Minimum Voltage.
      mask TypeOptions LoadType: Constant Z | constant I | constant P
      mask DialogControl ParameterTabVar0 Prompt: Parameters
      mask DialogControl ParameterTabVar1 Prompt: Type
      mask Display:
      | color('red');
      | A=[-210,-180,-170,-160,-147,-140,-130,-120,-110,-80,-50,-49,-45,-39,-33,-26,-21,-18,-17,-19,-22,-22,-26,-27,-25,-22,-16,-9,-3,2,6,6,4,1,1,-3,-4,-2,2,7,14,20,26,29,30,28,24,24,21,20,21,25,31,37,44,49,50,50,80];
      | B=[-41.5,-41.5,-63,-20,-63,-20,-63,-20,-41.5,-41.5,-41.5,-34,-26,-21,-20,-22,-28,-37,-47,-57,-63,-63,-54,-44,-34,-26,-21,-20,-22,-28,-37,-47,-57,-63,-63,-54,-44,-34,-26,-21,-20,-22,-28,-37,-47,-57,-63,-63,-54,-44,-34,-26,-21,-20,-22,-28,-37,-41.50,-41.5];
      | plot(A,B);
      | color('black');
      | port_label('LConn', 1, '+')
  7-8 1 : powerlib/Elements/Distributed Parameters Line  Phases=3  Frequency=60  Resistance=R_1  Inductance=L_1  Capacitance=C_1  Length=200*ft2km  x1=[437.061191479492 4173.08837477824 4174.13245807205;376.991118430775 376.991118430775 376.991118430775;1.69071767223413 -2.40388290733218 2.30847832203189]  x2=[437.235288764976 4176.95237464203 4179.02152463043;376.991118430775 376.991118430775 376.991118430775;1.69045403238691 -2.40441057475356 2.30795216962957]  x3=[2.63816882982582 185.713990703951 185.622300012898;376.991118430775 376.991118430775 376.991118430775;0.131473509127915 2.37835243770251 0.793227466590214]  x4=[2.86519793384983 186.144376680926 185.880699135539;376.991118430775 376.991118430775 376.991118430775;2.86040848214208 -0.931059442950243 -2.48100482524049]  x5=2.50829994562911e-07  V1=ones(3,3)  V2=ones(3,3)  I1=ones(3,3)  I2=ones(3,3)  nHarmo=1  Measurements=None
      settings: SourceProductName=Simscape Electrical
  70 : Subsystem
  70 Y PQ : Subsystem  mask(Single Phase ZIP Load){Vnom=1.0*2401.78, fnom=60, Pnom=20e3*a, Qnom=10e3*a, LoadType=constant P, Vlim=0.7}
      mask prompts: Vnom "Nominal Voltage Vn (Vrms)"; fnom "Nominal Frequency fn (Hz)"; Pnom "Nominal Active power (W)"; Qnom "Nominal Reactive power (VAR)"; LoadType "Load Type"; Vlim "Minimum voltage (pu)"
      mask help:
      | Notes:
      | Single Phase ZIP load model which gets converted to constant Z type if the voltage becomes lower than the Minimum Voltage.
      mask TypeOptions LoadType: Constant Z | constant I | constant P
      mask DialogControl ParameterTabVar0 Prompt: Parameters
      mask DialogControl ParameterTabVar1 Prompt: Type
      mask Display:
      | color('red');
      | A=[-210,-180,-170,-160,-147,-140,-130,-120,-110,-80,-50,-49,-45,-39,-33,-26,-21,-18,-17,-19,-22,-22,-26,-27,-25,-22,-16,-9,-3,2,6,6,4,1,1,-3,-4,-2,2,7,14,20,26,29,30,28,24,24,21,20,21,25,31,37,44,49,50,50,80];
      | B=[-41.5,-41.5,-63,-20,-63,-20,-63,-20,-41.5,-41.5,-41.5,-34,-26,-21,-20,-22,-28,-37,-47,-57,-63,-63,-54,-44,-34,-26,-21,-20,-22,-28,-37,-47,-57,-63,-63,-54,-44,-34,-26,-21,-20,-22,-28,-37,-47,-57,-63,-63,-54,-44,-34,-26,-21,-20,-22,-28,-37,-41.50,-41.5];
      | plot(A,B);
      | color('black');
      | port_label('LConn', 1, '+')
  70-71 1 : powerlib/Elements/Distributed Parameters Line  Phases=1  Frequency=60  Resistance=R_9(1,1)  Inductance=L_9(1,1)  Capacitance=C_9(1,1)  Length=275*ft2km  x1=[3458.20251991098;376.991118430775;-0.0100098122163506]  x2=[3458.20230905687;376.991118430775;-0.0100098905437716]  x3=[6.32911683819174;376.991118430775;-0.0101383942986067]  x4=[6.3360323625165;376.991118430775;-0.0100099113030933]  x5=3.4093273678088e-07  V1=[2.049e+04;377;-2.115]  V2=[2.048e+04;377;-2.115]  I1=[33.62;377;-2.106]  I2=[35.2;377;-2.126]  nHarmo=1  Measurements=None
      settings: SourceProductName=Simscape Electrical
  71 : Subsystem
  71 Y PQ : Subsystem  mask(Single Phase ZIP Load){Vnom=1.0*2401.78, fnom=60, Pnom=40e3*a, Qnom=20e3*a, LoadType=constant P, Vlim=0.7}
      mask prompts: Vnom "Nominal Voltage Vn (Vrms)"; fnom "Nominal Frequency fn (Hz)"; Pnom "Nominal Active power (W)"; Qnom "Nominal Reactive power (VAR)"; LoadType "Load Type"; Vlim "Minimum voltage (pu)"
      mask help:
      | Notes:
      | Single Phase ZIP load model which gets converted to constant Z type if the voltage becomes lower than the Minimum Voltage.
      mask TypeOptions LoadType: Constant Z | constant I | constant P
      mask DialogControl ParameterTabVar0 Prompt: Parameters
      mask DialogControl ParameterTabVar1 Prompt: Type
      mask Display:
      | color('red');
      | A=[-210,-180,-170,-160,-147,-140,-130,-120,-110,-80,-50,-49,-45,-39,-33,-26,-21,-18,-17,-19,-22,-22,-26,-27,-25,-22,-16,-9,-3,2,6,6,4,1,1,-3,-4,-2,2,7,14,20,26,29,30,28,24,24,21,20,21,25,31,37,44,49,50,50,80];
      | B=[-41.5,-41.5,-63,-20,-63,-20,-63,-20,-41.5,-41.5,-41.5,-34,-26,-21,-20,-22,-28,-37,-47,-57,-63,-63,-54,-44,-34,-26,-21,-20,-22,-28,-37,-47,-57,-63,-63,-54,-44,-34,-26,-21,-20,-22,-28,-37,-47,-57,-63,-63,-54,-44,-34,-26,-21,-20,-22,-28,-37,-41.50,-41.5];
      | plot(A,B);
      | color('black');
      | port_label('LConn', 1, '+')
  72 : powerlib/Measurements/Three-Phase V-I Measurement  VoltageMeasurement=phase-to-ground  SetLabelV=on  LabelV=V72  Vpu=off  VpuLL=off  CurrentMeasurement=no  SetLabelI=on  LabelI=I65  Ipu=off  Pbase=100e6  Vbase=24900  OutputType=Complex  PhasorSimulation=on  PSBequivalent=0
      settings: SourceProductName=Simscape Electrical
  72-73 11 : powerlib/Elements/Distributed Parameters Line  Phases=1  Frequency=60  Resistance=R_11(3,3)  Inductance=L_11(3,3)  Capacitance=C_11(3,3)  Length=275*ft2km  x1=[3457.92787126941;376.991118430775;2.08692690041761]  x2=[3457.9273372984;376.991118430775;2.08692663725521]  x3=[6.32169769704375;376.991118430775;2.08644711397849]  x4=[6.34244611528141;376.991118430775;2.08727653212239]  x5=3.4093273678088e-07  V1=[2.049e+04;377;-2.115]  V2=[2.048e+04;377;-2.115]  I1=[33.62;377;-2.106]  I2=[35.2;377;-2.126]  nHarmo=1  Measurements=None
      settings: SourceProductName=Simscape Electrical
  72-76 3 : powerlib/Elements/Distributed Parameters Line  Phases=3  Frequency=60  Resistance=R_3  Inductance=L_3  Capacitance=C_3  Length=200*ft2km  x1=[443.603864090973 4239.00541261997 4237.49079663195;376.991118430775 376.991118430775 376.991118430775;-0.417291527789523 0.205411561173557 1.77827887468897]  x2=[443.771981179146 4243.91322144233 4241.36748601179;376.991118430775 376.991118430775 376.991118430775;-0.417546145130738 0.204902957397948 1.777767989902]  x3=[2.55572535162177 185.762720922153 185.568598581744;376.991118430775 376.991118430775 376.991118430775;-1.97335170304628 -1.30055663688097 0.287395966034407]  x4=[2.79342105832593 185.818339349021 185.731692532979;376.991118430775 376.991118430775 376.991118430775;0.737563766900212 1.70635402662685 -3.02488183132338]  x5=2.50829994562911e-07  V1=ones(3,3)  V2=ones(3,3)  I1=ones(3,3)  I2=ones(3,3)  nHarmo=1  Measurements=None
      settings: SourceProductName=Simscape Electrical
  73 : Subsystem
  73 Y PQ : Subsystem  mask(Single Phase ZIP Load){Vnom=1.0*2401.78, fnom=60, Pnom=40e3*a, Qnom=20e3*a, LoadType=constant P, Vlim=0.7}
      mask prompts: Vnom "Nominal Voltage Vn (Vrms)"; fnom "Nominal Frequency fn (Hz)"; Pnom "Nominal Active power (W)"; Qnom "Nominal Reactive power (VAR)"; LoadType "Load Type"; Vlim "Minimum voltage (pu)"
      mask help:
      | Notes:
      | Single Phase ZIP load model which gets converted to constant Z type if the voltage becomes lower than the Minimum Voltage.
      mask TypeOptions LoadType: Constant Z | constant I | constant P
      mask DialogControl ParameterTabVar0 Prompt: Parameters
      mask DialogControl ParameterTabVar1 Prompt: Type
      mask Display:
      | color('red');
      | A=[-210,-180,-170,-160,-147,-140,-130,-120,-110,-80,-50,-49,-45,-39,-33,-26,-21,-18,-17,-19,-22,-22,-26,-27,-25,-22,-16,-9,-3,2,6,6,4,1,1,-3,-4,-2,2,7,14,20,26,29,30,28,24,24,21,20,21,25,31,37,44,49,50,50,80];
      | B=[-41.5,-41.5,-63,-20,-63,-20,-63,-20,-41.5,-41.5,-41.5,-34,-26,-21,-20,-22,-28,-37,-47,-57,-63,-63,-54,-44,-34,-26,-21,-20,-22,-28,-37,-47,-57,-63,-63,-54,-44,-34,-26,-21,-20,-22,-28,-37,-47,-57,-63,-63,-54,-44,-34,-26,-21,-20,-22,-28,-37,-41.50,-41.5];
      | plot(A,B);
      | color('black');
      | port_label('LConn', 1, '+')
  73-74 11 : powerlib/Elements/Distributed Parameters Line  Phases=1  Frequency=60  Resistance=R_11(3,3)  Inductance=L_11(3,3)  Capacitance=C_11(3,3)  Length=350*ft2km  x1=[3457.9273372984;376.991118430775;2.08689158399692]  x2=[3457.92687995695;376.991118430775;2.08689136198628]  x3=[6.3249917458279;376.991118430775;2.08654065369966]  x4=[6.33882122590306;376.991118430775;2.08707811687743]  x5=4.33914392266575e-07  V1=[2.049e+04;377;-2.115]  V2=[2.048e+04;377;-2.115]  I1=[33.62;377;-2.106]  I2=[35.2;377;-2.126]  nHarmo=1  Measurements=None
      settings: SourceProductName=Simscape Electrical
  74 : Subsystem
  74 Y Z : Subsystem  mask(Single Phase ZIP Load){Vnom=1.0*2401.78, fnom=60, Pnom=40e3*a, Qnom=20e3*a, LoadType=Constant Z, Vlim=0.7}
      mask prompts: Vnom "Nominal Voltage Vn (Vrms)"; fnom "Nominal Frequency fn (Hz)"; Pnom "Nominal Active power (W)"; Qnom "Nominal Reactive power (VAR)"; LoadType "Load Type"; Vlim "Minimum voltage (pu)"
      mask help:
      | Notes:
      | Single Phase ZIP load model which gets converted to constant Z type if the voltage becomes lower than the Minimum Voltage.
      mask TypeOptions LoadType: Constant Z | constant I | constant P
      mask DialogControl ParameterTabVar0 Prompt: Parameters
      mask DialogControl ParameterTabVar1 Prompt: Type
      mask Display:
      | color('red');
      | A=[-210,-180,-170,-160,-147,-140,-130,-120,-110,-80,-50,-49,-45,-39,-33,-26,-21,-18,-17,-19,-22,-22,-26,-27,-25,-22,-16,-9,-3,2,6,6,4,1,1,-3,-4,-2,2,7,14,20,26,29,30,28,24,24,21,20,21,25,31,37,44,49,50,50,80];
      | B=[-41.5,-41.5,-63,-20,-63,-20,-63,-20,-41.5,-41.5,-41.5,-34,-26,-21,-20,-22,-28,-37,-47,-57,-63,-63,-54,-44,-34,-26,-21,-20,-22,-28,-37,-47,-57,-63,-63,-54,-44,-34,-26,-21,-20,-22,-28,-37,-47,-57,-63,-63,-54,-44,-34,-26,-21,-20,-22,-28,-37,-41.50,-41.5];
      | plot(A,B);
      | color('black');
      | port_label('LConn', 1, '+')
  74-75 11 : powerlib/Elements/Distributed Parameters Line  Phases=1  Frequency=60  Resistance=R_11(3,3)  Inductance=L_11(3,3)  Capacitance=C_11(3,3)  Length=400*ft2km  x1=[3457.92687995695;376.991118430775;2.08686799314742]  x2=[3457.9265921816;376.991118430775;2.08686787382589]  x3=[6.32833885309252;376.991118430775;2.08668093174932]  x4=[6.33525343067953;376.991118430775;2.08686787381927]  x5=4.95902162590371e-07  V1=[2.049e+04;377;-2.115]  V2=[2.048e+04;377;-2.115]  I1=[33.62;377;-2.106]  I2=[35.2;377;-2.126]  nHarmo=1  Measurements=None
      settings: SourceProductName=Simscape Electrical
  75 : Subsystem
  75 Y PQ : Subsystem  mask(Single Phase ZIP Load){Vnom=1.0*2401.78, fnom=60, Pnom=40e3*a, Qnom=20e3*a, LoadType=constant P, Vlim=0.7}
      mask prompts: Vnom "Nominal Voltage Vn (Vrms)"; fnom "Nominal Frequency fn (Hz)"; Pnom "Nominal Active power (W)"; Qnom "Nominal Reactive power (VAR)"; LoadType "Load Type"; Vlim "Minimum voltage (pu)"
      mask help:
      | Notes:
      | Single Phase ZIP load model which gets converted to constant Z type if the voltage becomes lower than the Minimum Voltage.
      mask TypeOptions LoadType: Constant Z | constant I | constant P
      mask DialogControl ParameterTabVar0 Prompt: Parameters
      mask DialogControl ParameterTabVar1 Prompt: Type
      mask Display:
      | color('red');
      | A=[-210,-180,-170,-160,-147,-140,-130,-120,-110,-80,-50,-49,-45,-39,-33,-26,-21,-18,-17,-19,-22,-22,-26,-27,-25,-22,-16,-9,-3,2,6,6,4,1,1,-3,-4,-2,2,7,14,20,26,29,30,28,24,24,21,20,21,25,31,37,44,49,50,50,80];
      | B=[-41.5,-41.5,-63,-20,-63,-20,-63,-20,-41.5,-41.5,-41.5,-34,-26,-21,-20,-22,-28,-37,-47,-57,-63,-63,-54,-44,-34,-26,-21,-20,-22,-28,-37,-47,-57,-63,-63,-54,-44,-34,-26,-21,-20,-22,-28,-37,-47,-57,-63,-63,-54,-44,-34,-26,-21,-20,-22,-28,-37,-41.50,-41.5];
      | plot(A,B);
      | color('black');
      | port_label('LConn', 1, '+')
  76 : powerlib/Measurements/Three-Phase V-I Measurement  VoltageMeasurement=phase-to-ground  SetLabelV=on  LabelV=V76  Vpu=off  VpuLL=off  CurrentMeasurement=no  SetLabelI=on  LabelI=I65  Ipu=off  Pbase=100e6  Vbase=24900  OutputType=Complex  PhasorSimulation=on  PSBequivalent=0
      settings: SourceProductName=Simscape Electrical
  76 DI : Subsystem  mask(Three Phase Delta ZIP Load (Phasor)){Vnom=4160, fnom=60, Pnom=[105 70  70]*1e3*a, Qnom=[80 50 50]*1e3*a, LoadType=Constant I, Vlim=0.7}
      mask prompts: Vnom "Nominal Ph-Ph Voltage (Vrms)"; fnom "Nominal Frequency fn (Hz)"; Pnom "Nominal Per Phase Active Power [Pab Pbc Pca] (W)"; Qnom "Nominal Per Phase Reactive Power [Qab Qbc Qca] (VAR)"; LoadType "Load Type"; Vlim "Minimum Voltage (pu)"
      mask help:
      | Notes:
      | Three Phase Delta Connected ZIP load model which gets converted to constant Z type if the voltage becomes lower than the Minimum Voltage.
      mask TypeOptions LoadType: Constant Z | Constant I | Constant P
      mask DialogControl ParameterTabVar0 Prompt: Parameters
      mask DialogControl ParameterTabVar01 Prompt: Type
      mask Display:
      | color('red');
      | %load figure 0deg
      | A=[-210,-180,-170,-160,-147,-140,-130,-120,-110,-80,-50,-49,-45,-39,-33,-26,-21,-18,-17,-19,-22,-22,-26,-27,-25,-22,-16,-9,-3,2,6,6,4,1,1,-3,-4,-2,2,7,14,20,26,29,30,28,24,24,21,20,21,25,31,37,44,49,50,50,80];
      | B=[-41.5,-41.5,-63,-20,-63,-20,-63,-20,-41.5,-41.5,-41.5,-34,-26,-21,-20,-22,-28,-37,-47,-57,-63,-63,-54,-44,-34,-26,-21,-20,-22,-28,-37,-47,-57,-63,-63,-54,-44,-34,-26,-21,-20,-22,-28,-37,-47,-57,-63,-63,-54,-44,-34,-26,-21,-20,-22,-28,-37,-41.50,-41.5];
      | plot(A,B);
      | 
      | %load figure 0deg inverted
      | A1=[-80,-50,-49,-45,-39,-33,-26,-21,-18,-17,-19,-22,-22,-26,-27,-25,-22,-16,-9,-3,2,6,6,4,1,1,-3,-4,-2,2,7,14,20,26,29,30,28,24,24,21,20,21,25,31,37,44,49,50,50,80,110,120,130,143,150,160,170,180,210];
      | B1=[-41.5,-41.5,-34,-26,-21,-20,-22,-28,-37,-47,-57,-63,-63,-54,-44,-34,-26,-21,-20,-22,-28,-37,-47,-57,-63,-63,-54,-44,-34,-26,-21,-20,-22,-28,-37,-47,-57,-63,-63,-54,-44,-34,-26,-21,-20,-22,-28,-37,-41.5,-41.5,-41.5,-63,-20,-63,-20,-63,-20,-41.5,-41.5];
      | 
      | 
      | %load figure -120deg
      | c=1*exp(sqrt(-1)*(-60*pi/180));
      | l=A1+j*B1;
      | m=l*c;
      | E=real(m);F=imag(m);
      | E=E+10.94;F=F+161.1;
      | plot(E,F);
      | 
      | %load figure +120deg
      | c=1*exp(sqrt(-1)*(60*pi/180));
      | l=A1+j*B1;
      | m=l*c;
      | G=real(m);
      | H=imag(m);
      | G=G-205.94;H=H+48.53;
      | plot(G,H);
      | 
      | color('black');
      | port_label('LConn', 1, 'A')
      | port_label('LConn', 2, 'B')
      | port_label('LConn', 3, 'C')
  76-77 6 : powerlib/Elements/Distributed Parameters Line  Phases=3  Frequency=60  Resistance=R_6  Inductance=L_6  Capacitance=C_6  Length=400*ft2km  x1=[446.384445889856 4247.15074660521 4238.09513020516;376.991118430775 376.991118430775 376.991118430775;-1.70732709547682 2.39268744138778 -2.32148662736559]  x2=[446.708315230087 4253.37226513741 4245.94301543386;376.991118430775 376.991118430775 376.991118430775;-1.70745996497188 2.39187382352043 -2.3223048957353]  x3=[2.31313078968722 149.040941843884 148.823439975539;376.991118430775 376.991118430775 376.991118430775;-2.82665882431221 0.925064003023854 2.46999535154546]  x4=[2.08768945304178 149.135236017482 148.936355332857;376.991118430775 376.991118430775 376.991118430775;-0.215476803869229 -2.42975544046229 -0.839757581452542]  x5=5.01659989125821e-07  V1=ones(3,3)  V2=ones(3,3)  I1=ones(3,3)  I2=ones(3,3)  nHarmo=1  Measurements=None
      settings: SourceProductName=Simscape Electrical
  76-86 3 : powerlib/Elements/Distributed Parameters Line  Phases=3  Frequency=60  Resistance=R_3  Inductance=L_3  Capacitance=C_3  Length=700*ft2km  x1=[443.771981179146 4243.91322144233 4241.36748601179;376.991118430775 376.991118430775 376.991118430775;-0.417782546831203 0.204707671564561 1.77757185094247]  x2=[443.88055636918 4247.33488875513 4244.07411041575;376.991118430775 376.991118430775 376.991118430775;-0.417958135737355 0.204355133344671 1.777218101003]  x3=[0.667607723864108 38.9520896634416 40.0606476991273;376.991118430775 376.991118430775 376.991118430775;-1.21675113749177 -1.03980570567268 0.610865804349187]  x4=[0.848541437182649 38.9628371444185 40.1184199035977;376.991118430775 376.991118430775 376.991118430775;0.180810858335731 1.44778159303285 2.94029792103028]  x5=8.77904980970188e-07  V1=ones(3,3)  V2=ones(3,3)  I1=ones(3,3)  I2=ones(3,3)  nHarmo=1  Measurements=None
      settings: SourceProductName=Simscape Electrical
  77 : powerlib/Measurements/Three-Phase V-I Measurement  VoltageMeasurement=phase-to-ground  SetLabelV=on  LabelV=V77  Vpu=off  VpuLL=off  CurrentMeasurement=no  SetLabelI=on  LabelI=I65  Ipu=off  Pbase=100e6  Vbase=24900  OutputType=Complex  PhasorSimulation=on  PSBequivalent=0
      settings: SourceProductName=Simscape Electrical
  77 Y PQ : Subsystem  mask(Single Phase ZIP Load){Vnom=1.0*2401.78, fnom=60, Pnom=40e3*a, Qnom=20e3*a, LoadType=constant P, Vlim=0.7}
      mask prompts: Vnom "Nominal Voltage Vn (Vrms)"; fnom "Nominal Frequency fn (Hz)"; Pnom "Nominal Active power (W)"; Qnom "Nominal Reactive power (VAR)"; LoadType "Load Type"; Vlim "Minimum voltage (pu)"
      mask help:
      | Notes:
      | Single Phase ZIP load model which gets converted to constant Z type if the voltage becomes lower than the Minimum Voltage.
      mask TypeOptions LoadType: Constant Z | constant I | constant P
      mask DialogControl ParameterTabVar0 Prompt: Parameters
      mask DialogControl ParameterTabVar1 Prompt: Type
      mask Display:
      | color('red');
      | A=[-210,-180,-170,-160,-147,-140,-130,-120,-110,-80,-50,-49,-45,-39,-33,-26,-21,-18,-17,-19,-22,-22,-26,-27,-25,-22,-16,-9,-3,2,6,6,4,1,1,-3,-4,-2,2,7,14,20,26,29,30,28,24,24,21,20,21,25,31,37,44,49,50,50,80];
      | B=[-41.5,-41.5,-63,-20,-63,-20,-63,-20,-41.5,-41.5,-41.5,-34,-26,-21,-20,-22,-28,-37,-47,-57,-63,-63,-54,-44,-34,-26,-21,-20,-22,-28,-37,-47,-57,-63,-63,-54,-44,-34,-26,-21,-20,-22,-28,-37,-47,-57,-63,-63,-54,-44,-34,-26,-21,-20,-22,-28,-37,-41.50,-41.5];
      | plot(A,B);
      | color('black');
      | port_label('LConn', 1, '+')
  77-78 6 : powerlib/Elements/Distributed Parameters Line  Phases=3  Frequency=60  Resistance=R_6  Inductance=L_6  Capacitance=C_6  Length=100*ft2km  x1=[446.708315230087 4253.37226513741 4245.94301543386;376.991118430775 376.991118430775 376.991118430775;-1.7073181239516 2.39199150689615 -2.32218772423526]  x2=[446.789337272588 4254.92807311533 4247.90542101468;376.991118430775 376.991118430775 376.991118430775;-1.70735118253153 2.39178847596586 -2.32239180854507]  x3=[2.3148996796593 149.059056681203 148.837000070333;376.991118430775 376.991118430775 376.991118430775;-2.82575758309762 0.92533149133977 2.47028137280392]  x4=[2.08835796026859 149.137376152722 148.93688099938;376.991118430775 376.991118430775 376.991118430775;-0.21445899714484 -2.42967997298039 -0.839665351924848]  x5=1.25414997281455e-07  V1=ones(3,3)  V2=ones(3,3)  I1=ones(3,3)  I2=ones(3,3)  nHarmo=1  Measurements=None
      settings: SourceProductName=Simscape Electrical
  78 : powerlib/Measurements/Three-Phase V-I Measurement  VoltageMeasurement=phase-to-ground  SetLabelV=on  LabelV=V78  Vpu=off  VpuLL=off  CurrentMeasurement=no  SetLabelI=on  LabelI=I65  Ipu=off  Pbase=100e6  Vbase=24900  OutputType=Complex  PhasorSimulation=on  PSBequivalent=0
      settings: SourceProductName=Simscape Electrical
  78-79 6 : powerlib/Elements/Distributed Parameters Line  Phases=3  Frequency=60  Resistance=R_6  Inductance=L_6  Capacitance=C_6  Length=225*ft2km  x1=[446.789337272588 4254.92807311533 4247.90542101468;376.991118430775 376.991118430775 376.991118430775;-1.70741028295664 2.39173944122598 -2.32244063000341]  x2=[446.78951068725 4254.92810203783 4247.9053731557;376.991118430775 376.991118430775 376.991118430775;-1.70741038564338 2.39173942689536 -2.32244063684057]  x3=[0.587502385997275 15.8811748663567 12.5194496230542;376.991118430775 376.991118430775 376.991118430775;-1.71093828474837 2.39156757223971 -2.32240545168662]  x4=[0.586998133345675 15.8840931801504 12.5222634376029;376.991118430775 376.991118430775 376.991118430775;-1.70398578079494 2.39182300880936 -2.3225636768468]  x5=2.82183743883275e-07  V1=ones(3,3)  V2=ones(3,3)  I1=ones(3,3)  I2=ones(3,3)  nHarmo=1  Measurements=None
      settings: SourceProductName=Simscape Electrical
  78-80 6 : powerlib/Elements/Distributed Parameters Line  Phases=3  Frequency=60  Resistance=R_6  Inductance=L_6  Capacitance=C_6  Length=475*ft2km  x1=[446.789337272588 4254.92807311533 4247.90542101468;376.991118430775 376.991118430775 376.991118430775;-1.70752848380688 2.39164137174622 -2.32253827292011]  x2=[447.173813706657 4262.32036542174 4257.22923513584;376.991118430775 376.991118430775 376.991118430775;-1.70768511463596 2.39067904563094 -2.32350507654625]  x3=[2.31287853544668 149.053598586761 148.835298005855;376.991118430775 376.991118430775 376.991118430775;-2.82560195810998 0.925230816454334 2.47018037739859]  x4=[2.08605277952876 149.113254401006 148.920432966409;376.991118430775 376.991118430775 376.991118430775;-0.215078442788336 -2.4300144200522 -0.839993119051423]  x5=5.95721237086913e-07  V1=ones(3,3)  V2=ones(3,3)  I1=ones(3,3)  I2=ones(3,3)  nHarmo=1  Measurements=None
      settings: SourceProductName=Simscape Electrical
  79 : powerlib/Measurements/Three-Phase V-I Measurement  VoltageMeasurement=phase-to-ground  SetLabelV=on  LabelV=V79  Vpu=off  VpuLL=off  CurrentMeasurement=no  SetLabelI=on  LabelI=I65  Ipu=off  Pbase=100e6  Vbase=24900  OutputType=Complex  PhasorSimulation=on  PSBequivalent=0
      settings: SourceProductName=Simscape Electrical
  79 Y Z : Subsystem  mask(Single Phase ZIP Load){Vnom=1.0*2401.78, fnom=60, Pnom=40e3*a, Qnom=20e3*a, LoadType=Constant Z, Vlim=0.7}
      mask prompts: Vnom "Nominal Voltage Vn (Vrms)"; fnom "Nominal Frequency fn (Hz)"; Pnom "Nominal Active power (W)"; Qnom "Nominal Reactive power (VAR)"; LoadType "Load Type"; Vlim "Minimum voltage (pu)"
      mask help:
      | Notes:
      | Single Phase ZIP load model which gets converted to constant Z type if the voltage becomes lower than the Minimum Voltage.
      mask TypeOptions LoadType: Constant Z | constant I | constant P
      mask DialogControl ParameterTabVar0 Prompt: Parameters
      mask DialogControl ParameterTabVar1 Prompt: Type
      mask Display:
      | color('red');
      | A=[-210,-180,-170,-160,-147,-140,-130,-120,-110,-80,-50,-49,-45,-39,-33,-26,-21,-18,-17,-19,-22,-22,-26,-27,-25,-22,-16,-9,-3,2,6,6,4,1,1,-3,-4,-2,2,7,14,20,26,29,30,28,24,24,21,20,21,25,31,37,44,49,50,50,80];
      | B=[-41.5,-41.5,-63,-20,-63,-20,-63,-20,-41.5,-41.5,-41.5,-34,-26,-21,-20,-22,-28,-37,-47,-57,-63,-63,-54,-44,-34,-26,-21,-20,-22,-28,-37,-47,-57,-63,-63,-54,-44,-34,-26,-21,-20,-22,-28,-37,-47,-57,-63,-63,-54,-44,-34,-26,-21,-20,-22,-28,-37,-41.50,-41.5];
      | plot(A,B);
      | color('black');
      | port_label('LConn', 1, '+')
  8 : powerlib/Measurements/Three-Phase V-I Measurement  VoltageMeasurement=phase-to-ground  SetLabelV=on  LabelV=V8  Vpu=off  VpuLL=off  CurrentMeasurement=no  SetLabelI=on  LabelI=I800  Ipu=off  Pbase=100e6  Vbase=24900  OutputType=Complex  PhasorSimulation=on  PSBequivalent=0
      settings: SourceProductName=Simscape Electrical
  8-12 10 : powerlib/Elements/Distributed Parameters Line  Phases=1  Frequency=60  Resistance=R_10(2,2)  Inductance=L_10(2,2)  Capacitance=C_10(2,2)  Length=225*ft2km  x1=[3411.88074696942;376.991118430775;-2.09646476450029]  x2=[3411.88057257925;376.991118430775;-2.09646482737709]  x3=[6.24444782059493;376.991118430775;-2.09656998853092]  x4=[6.25127089305498;376.991118430775;-2.09646482327163]  x5=2.78944966457084e-07  V1=[2.049e+04;377;-2.115]  V2=[2.048e+04;377;-2.115]  I1=[33.62;377;-2.106]  I2=[35.2;377;-2.126]  nHarmo=1  Measurements=None
      settings: SourceProductName=Simscape Electrical
  8-13 1 : powerlib/Elements/Distributed Parameters Line  Phases=3  Frequency=60  Resistance=R_1  Inductance=L_1  Capacitance=C_1  Length=300*ft2km  x1=[437.235288764976 4176.95237464203 4179.02152463043;376.991118430775 376.991118430775 376.991118430775;1.69040675204681 -2.40444980254547 2.30791311246289]  x2=[437.497229956295 4182.75074305891 4186.35705934251;376.991118430775 376.991118430775 376.991118430775;1.69001080031079 -2.40523940739788 2.30712626387474]  x3=[2.64543593995697 185.723047518056 185.620769431718;376.991118430775 376.991118430775 376.991118430775;0.13120297127167 2.37843769477008 0.793290525769722]  x4=[2.87193543179294 186.131842174419 185.862790258988;376.991118430775 376.991118430775 376.991118430775;2.86095391767615 -0.931169264144098 -2.48114233339232]  x5=3.76244991844366e-07  V1=ones(3,3)  V2=ones(3,3)  I1=ones(3,3)  I2=ones(3,3)  nHarmo=1  Measurements=None
      settings: SourceProductName=Simscape Electrical
  8-9 9 : powerlib/Elements/Distributed Parameters Line  Phases=1  Frequency=60  Resistance=R_9(1,1)  Inductance=L_9(1,1)  Capacitance=C_9(1,1)  Length=225*ft2km  x1=[3412.46953939907;376.991118430775;-0.00327369130412523]  x2=[3412.46894024718;376.991118430775;-0.00327397129193977]  x3=[6.23528941320439;376.991118430775;-0.00381236041094156]  x4=[6.26258637607173;376.991118430775;-0.00284258280469495]  x5=2.78944966457084e-07  V1=[2.049e+04;377;-2.115]  V2=[2.048e+04;377;-2.115]  I1=[33.62;377;-2.106]  I2=[35.2;377;-2.126]  nHarmo=1  Measurements=None
      settings: SourceProductName=Simscape Electrical
  80 : powerlib/Measurements/Three-Phase V-I Measurement  VoltageMeasurement=phase-to-ground  SetLabelV=on  LabelV=V80  Vpu=off  VpuLL=off  CurrentMeasurement=no  SetLabelI=on  LabelI=I65  Ipu=off  Pbase=100e6  Vbase=24900  OutputType=Complex  PhasorSimulation=on  PSBequivalent=0
      settings: SourceProductName=Simscape Electrical
  80 Y PQ : Subsystem  mask(Single Phase ZIP Load){Vnom=1.0*2401.78, fnom=60, Pnom=40e3*a, Qnom=20e3*a, LoadType=constant P, Vlim=0.7}
      mask prompts: Vnom "Nominal Voltage Vn (Vrms)"; fnom "Nominal Frequency fn (Hz)"; Pnom "Nominal Active power (W)"; Qnom "Nominal Reactive power (VAR)"; LoadType "Load Type"; Vlim "Minimum voltage (pu)"
      mask help:
      | Notes:
      | Single Phase ZIP load model which gets converted to constant Z type if the voltage becomes lower than the Minimum Voltage.
      mask TypeOptions LoadType: Constant Z | constant I | constant P
      mask DialogControl ParameterTabVar0 Prompt: Parameters
      mask DialogControl ParameterTabVar1 Prompt: Type
      mask Display:
      | color('red');
      | A=[-210,-180,-170,-160,-147,-140,-130,-120,-110,-80,-50,-49,-45,-39,-33,-26,-21,-18,-17,-19,-22,-22,-26,-27,-25,-22,-16,-9,-3,2,6,6,4,1,1,-3,-4,-2,2,7,14,20,26,29,30,28,24,24,21,20,21,25,31,37,44,49,50,50,80];
      | B=[-41.5,-41.5,-63,-20,-63,-20,-63,-20,-41.5,-41.5,-41.5,-34,-26,-21,-20,-22,-28,-37,-47,-57,-63,-63,-54,-44,-34,-26,-21,-20,-22,-28,-37,-47,-57,-63,-63,-54,-44,-34,-26,-21,-20,-22,-28,-37,-47,-57,-63,-63,-54,-44,-34,-26,-21,-20,-22,-28,-37,-41.50,-41.5];
      | plot(A,B);
      | color('black');
      | port_label('LConn', 1, '+')
  80-81 6 : powerlib/Elements/Distributed Parameters Line  Phases=3  Frequency=60  Resistance=R_6  Inductance=L_6  Capacitance=C_6  Length=475*ft2km  x1=[447.173813706657 4262.32036542174 4257.22923513584;376.991118430775 376.991118430775 376.991118430775;-1.70768511463596 2.39067904563094 -2.32350507654625]  x2=[447.558545241107 4269.71646964566 4266.55689911704;376.991118430775 376.991118430775 376.991118430775;-1.70784085516811 2.38972006987007 -2.32446759768501]  x3=[2.31461376022287 149.069237156244 148.846930715531;376.991118430775 376.991118430775 376.991118430775;-2.82481323641129 0.92540659094351 2.47037639821346]  x4=[2.08652012093527 149.098555571656 148.90767505772;376.991118430775 376.991118430775 376.991118430775;-0.214392917338172 -2.4302106362852 -0.840168789742534]  x5=5.95721237086913e-07  V1=ones(3,3)  V2=ones(3,3)  I1=ones(3,3)  I2=ones(3,3)  nHarmo=1  Measurements=None
      settings: SourceProductName=Simscape Electrical
  81 : powerlib/Measurements/Three-Phase V-I Measurement  VoltageMeasurement=phase-to-ground  SetLabelV=on  LabelV=V81  Vpu=off  VpuLL=off  CurrentMeasurement=no  SetLabelI=on  LabelI=I65  Ipu=off  Pbase=100e6  Vbase=24900  OutputType=Complex  PhasorSimulation=on  PSBequivalent=0
      settings: SourceProductName=Simscape Electrical
  81-82 6 : powerlib/Elements/Distributed Parameters Line  Phases=3  Frequency=60  Resistance=R_6  Inductance=L_6  Capacitance=C_6  Length=250*ft2km  x1=[447.558545241107 4269.71646964566 4266.55689911704;376.991118430775 376.991118430775 376.991118430775;-1.7077344744029 2.38980833240185 -2.32437971905998]  x2=[447.76131573354 4273.61073521162 4271.46763895985;376.991118430775 376.991118430775 376.991118430775;-1.70781704658208 2.38930499106889 -2.32488460938097]  x3=[2.31754566227496 149.087773718001 148.859484099833;376.991118430775 376.991118430775 376.991118430775;-2.82602249898088 0.92571387483025 2.47064272168018]  x4=[2.09057690478236 149.092622829289 148.902002237202;376.991118430775 376.991118430775 376.991118430775;-0.215223227172845 -2.43018652866408 -0.840186595331353]  x5=3.13537493203638e-07  V1=ones(3,3)  V2=ones(3,3)  I1=ones(3,3)  I2=ones(3,3)  nHarmo=1  Measurements=None
      settings: SourceProductName=Simscape Electrical
  81-84 11 : powerlib/Elements/Distributed Parameters Line  Phases=1  Frequency=60  Resistance=R_11(3,3)  Inductance=L_11(3,3)  Capacitance=C_11(3,3)  Length=675*ft2km  x1=[3485.10782753314;376.991118430775;2.08206055128908]  x2=[3485.10706061029;376.991118430775;2.08206008857745]  x3=[6.37399219596277;376.991118430775;2.08152243903149]  x4=[6.38792850214472;376.991118430775;2.08228186765333]  x5=8.36834899371251e-07  V1=[2.049e+04;377;-2.115]  V2=[2.048e+04;377;-2.115]  I1=[33.62;377;-2.106]  I2=[35.2;377;-2.126]  nHarmo=1  Measurements=None
      settings: SourceProductName=Simscape Electrical
  82 : powerlib/Measurements/Three-Phase V-I Measurement  VoltageMeasurement=phase-to-ground  SetLabelV=on  LabelV=V82  Vpu=off  VpuLL=off  CurrentMeasurement=no  SetLabelI=on  LabelI=I65  Ipu=off  Pbase=100e6  Vbase=24900  OutputType=Complex  PhasorSimulation=on  PSBequivalent=0
      settings: SourceProductName=Simscape Electrical
  82 Y PQ : Subsystem  mask(Single Phase ZIP Load){Vnom=1.0*2401.78, fnom=60, Pnom=40e3*a, Qnom=20e3*a, LoadType=constant P, Vlim=0.7}
      mask prompts: Vnom "Nominal Voltage Vn (Vrms)"; fnom "Nominal Frequency fn (Hz)"; Pnom "Nominal Active power (W)"; Qnom "Nominal Reactive power (VAR)"; LoadType "Load Type"; Vlim "Minimum voltage (pu)"
      mask help:
      | Notes:
      | Single Phase ZIP load model which gets converted to constant Z type if the voltage becomes lower than the Minimum Voltage.
      mask TypeOptions LoadType: Constant Z | constant I | constant P
      mask DialogControl ParameterTabVar0 Prompt: Parameters
      mask DialogControl ParameterTabVar1 Prompt: Type
      mask Display:
      | color('red');
      | A=[-210,-180,-170,-160,-147,-140,-130,-120,-110,-80,-50,-49,-45,-39,-33,-26,-21,-18,-17,-19,-22,-22,-26,-27,-25,-22,-16,-9,-3,2,6,6,4,1,1,-3,-4,-2,2,7,14,20,26,29,30,28,24,24,21,20,21,25,31,37,44,49,50,50,80];
      | B=[-41.5,-41.5,-63,-20,-63,-20,-63,-20,-41.5,-41.5,-41.5,-34,-26,-21,-20,-22,-28,-37,-47,-57,-63,-63,-54,-44,-34,-26,-21,-20,-22,-28,-37,-47,-57,-63,-63,-54,-44,-34,-26,-21,-20,-22,-28,-37,-47,-57,-63,-63,-54,-44,-34,-26,-21,-20,-22,-28,-37,-41.50,-41.5];
      | plot(A,B);
      | color('black');
      | port_label('LConn', 1, '+')
  82-83 6 : powerlib/Elements/Distributed Parameters Line  Phases=3  Frequency=60  Resistance=R_6  Inductance=L_6  Capacitance=C_6  Length=250*ft2km  x1=[447.76131573354 4273.61073521162 4271.46763895985;376.991118430775 376.991118430775 376.991118430775;-1.70781704658208 2.38930499106889 -2.32488460938097]  x2=[447.96389223412 4277.50602656071 4276.37949616883;376.991118430775 376.991118430775 376.991118430775;-1.7078994261796 2.38880258517977 -2.32538833011271]  x3=[2.31571640876567 149.094580376711 148.867450013681;376.991118430775 376.991118430775 376.991118430775;-2.82563110355651 0.925816921522537 2.47074537935095]  x4=[2.0884852979647 149.083160927355 148.897116758928;376.991118430775 376.991118430775 376.991118430775;-0.215550338025066 -2.43028154023578 -0.840277470131045]  x5=3.13537493203638e-07  V1=ones(3,3)  V2=ones(3,3)  I1=ones(3,3)  I2=ones(3,3)  nHarmo=1  Measurements=None
      settings: SourceProductName=Simscape Electrical
  83 : powerlib/Measurements/Three-Phase V-I Measurement  VoltageMeasurement=phase-to-ground  SetLabelV=on  LabelV=V83  Vpu=off  VpuLL=off  CurrentMeasurement=no  SetLabelI=on  LabelI=I65  Ipu=off  Pbase=100e6  Vbase=24900  OutputType=Complex  PhasorSimulation=on  PSBequivalent=0
      settings: SourceProductName=Simscape Electrical
  83 Y CAP : powerlib/Elements/Three-Phase Series RLC Load  LConnTagsString=A|B|C  Configuration=Y (grounded)  NominalVoltage=120e3  Vabc=[ 1.0 1.0 1.0]*2401.78  Vabcp=[1e3 1e3 1e3]  NominalFrequency=60  UnbalancedPower=on  ActivePower=1e+006  InductivePower=0  CapacitivePower=0  Pabc=[0 0 0 ]*1e3  QLabc=[0 0 0 ]*1e3  QCabc=[200 200 200]*1e3*a  Pabcp=[10e3 9e3 11e3]  QLabcp=[100 90 110]  QCabcp=[100 90 110]  Measurements=None  LoadType=constant Z
      settings: SourceProductName=Simscape Electrical
  83 Y PQ : Subsystem  mask(Single Phase ZIP Load){Vnom=1.0*2401.78, fnom=60, Pnom=20e3*a, Qnom=10e3*a, LoadType=constant P, Vlim=0.7}
      mask prompts: Vnom "Nominal Voltage Vn (Vrms)"; fnom "Nominal Frequency fn (Hz)"; Pnom "Nominal Active power (W)"; Qnom "Nominal Reactive power (VAR)"; LoadType "Load Type"; Vlim "Minimum voltage (pu)"
      mask help:
      | Notes:
      | Single Phase ZIP load model which gets converted to constant Z type if the voltage becomes lower than the Minimum Voltage.
      mask TypeOptions LoadType: Constant Z | constant I | constant P
      mask DialogControl ParameterTabVar0 Prompt: Parameters
      mask DialogControl ParameterTabVar1 Prompt: Type
      mask Display:
      | color('red');
      | A=[-210,-180,-170,-160,-147,-140,-130,-120,-110,-80,-50,-49,-45,-39,-33,-26,-21,-18,-17,-19,-22,-22,-26,-27,-25,-22,-16,-9,-3,2,6,6,4,1,1,-3,-4,-2,2,7,14,20,26,29,30,28,24,24,21,20,21,25,31,37,44,49,50,50,80];
      | B=[-41.5,-41.5,-63,-20,-63,-20,-63,-20,-41.5,-41.5,-41.5,-34,-26,-21,-20,-22,-28,-37,-47,-57,-63,-63,-54,-44,-34,-26,-21,-20,-22,-28,-37,-47,-57,-63,-63,-54,-44,-34,-26,-21,-20,-22,-28,-37,-47,-57,-63,-63,-54,-44,-34,-26,-21,-20,-22,-28,-37,-41.50,-41.5];
      | plot(A,B);
      | color('black');
      | port_label('LConn', 1, '+')
  84 : Subsystem
  84 Y PQ : Subsystem  mask(Single Phase ZIP Load){Vnom=1.0*2401.78, fnom=60, Pnom=20e3*a, Qnom=10e3*a, LoadType=constant P, Vlim=0.7}
      mask prompts: Vnom "Nominal Voltage Vn (Vrms)"; fnom "Nominal Frequency fn (Hz)"; Pnom "Nominal Active power (W)"; Qnom "Nominal Reactive power (VAR)"; LoadType "Load Type"; Vlim "Minimum voltage (pu)"
      mask help:
      | Notes:
      | Single Phase ZIP load model which gets converted to constant Z type if the voltage becomes lower than the Minimum Voltage.
      mask TypeOptions LoadType: Constant Z | constant I | constant P
      mask DialogControl ParameterTabVar0 Prompt: Parameters
      mask DialogControl ParameterTabVar1 Prompt: Type
      mask Display:
      | color('red');
      | A=[-210,-180,-170,-160,-147,-140,-130,-120,-110,-80,-50,-49,-45,-39,-33,-26,-21,-18,-17,-19,-22,-22,-26,-27,-25,-22,-16,-9,-3,2,6,6,4,1,1,-3,-4,-2,2,7,14,20,26,29,30,28,24,24,21,20,21,25,31,37,44,49,50,50,80];
      | B=[-41.5,-41.5,-63,-20,-63,-20,-63,-20,-41.5,-41.5,-41.5,-34,-26,-21,-20,-22,-28,-37,-47,-57,-63,-63,-54,-44,-34,-26,-21,-20,-22,-28,-37,-47,-57,-63,-63,-54,-44,-34,-26,-21,-20,-22,-28,-37,-47,-57,-63,-63,-54,-44,-34,-26,-21,-20,-22,-28,-37,-41.50,-41.5];
      | plot(A,B);
      | color('black');
      | port_label('LConn', 1, '+')
  84-85 11 : powerlib/Elements/Distributed Parameters Line  Phases=1  Frequency=60  Resistance=R_11(3,3)  Inductance=L_11(3,3)  Capacitance=C_11(3,3)  Length=475*ft2km  x1=[3485.10706061029;376.991118430775;2.0821535639329]  x2=[3485.10672976017;376.991118430775;2.08215341839999]  x3=[6.3779158461585;376.991118430775;2.08193141983285]  x4=[6.38488447451625;376.991118430775;2.08215342515849]  x5=5.88883818076066e-07  V1=[2.049e+04;377;-2.115]  V2=[2.048e+04;377;-2.115]  I1=[33.62;377;-2.106]  I2=[35.2;377;-2.126]  nHarmo=1  Measurements=None
      settings: SourceProductName=Simscape Electrical
  85 : Subsystem
  85 Y PQ : Subsystem  mask(Single Phase ZIP Load){Vnom=1.0*2401.78, fnom=60, Pnom=40e3*a, Qnom=20e3*a, LoadType=constant P, Vlim=0.7}
      mask prompts: Vnom "Nominal Voltage Vn (Vrms)"; fnom "Nominal Frequency fn (Hz)"; Pnom "Nominal Active power (W)"; Qnom "Nominal Reactive power (VAR)"; LoadType "Load Type"; Vlim "Minimum voltage (pu)"
      mask help:
      | Notes:
      | Single Phase ZIP load model which gets converted to constant Z type if the voltage becomes lower than the Minimum Voltage.
      mask TypeOptions LoadType: Constant Z | constant I | constant P
      mask DialogControl ParameterTabVar0 Prompt: Parameters
      mask DialogControl ParameterTabVar1 Prompt: Type
      mask Display:
      | color('red');
      | A=[-210,-180,-170,-160,-147,-140,-130,-120,-110,-80,-50,-49,-45,-39,-33,-26,-21,-18,-17,-19,-22,-22,-26,-27,-25,-22,-16,-9,-3,2,6,6,4,1,1,-3,-4,-2,2,7,14,20,26,29,30,28,24,24,21,20,21,25,31,37,44,49,50,50,80];
      | B=[-41.5,-41.5,-63,-20,-63,-20,-63,-20,-41.5,-41.5,-41.5,-34,-26,-21,-20,-22,-28,-37,-47,-57,-63,-63,-54,-44,-34,-26,-21,-20,-22,-28,-37,-47,-57,-63,-63,-54,-44,-34,-26,-21,-20,-22,-28,-37,-47,-57,-63,-63,-54,-44,-34,-26,-21,-20,-22,-28,-37,-41.50,-41.5];
      | plot(A,B);
      | color('black');
      | port_label('LConn', 1, '+')
  86 : powerlib/Measurements/Three-Phase V-I Measurement  VoltageMeasurement=phase-to-ground  SetLabelV=on  LabelV=V86  Vpu=off  VpuLL=off  CurrentMeasurement=no  SetLabelI=on  LabelI=I65  Ipu=off  Pbase=100e6  Vbase=24900  OutputType=Complex  PhasorSimulation=on  PSBequivalent=0
      settings: SourceProductName=Simscape Electrical
  86 Y PQ : Subsystem  mask(Single Phase ZIP Load){Vnom=1.0*2401.78, fnom=60, Pnom=20e3*a, Qnom=10e3*a, LoadType=constant P, Vlim=0.7}
      mask prompts: Vnom "Nominal Voltage Vn (Vrms)"; fnom "Nominal Frequency fn (Hz)"; Pnom "Nominal Active power (W)"; Qnom "Nominal Reactive power (VAR)"; LoadType "Load Type"; Vlim "Minimum voltage (pu)"
      mask help:
      | Notes:
      | Single Phase ZIP load model which gets converted to constant Z type if the voltage becomes lower than the Minimum Voltage.
      mask TypeOptions LoadType: Constant Z | constant I | constant P
      mask DialogControl ParameterTabVar0 Prompt: Parameters
      mask DialogControl ParameterTabVar1 Prompt: Type
      mask Display:
      | color('red');
      | A=[-210,-180,-170,-160,-147,-140,-130,-120,-110,-80,-50,-49,-45,-39,-33,-26,-21,-18,-17,-19,-22,-22,-26,-27,-25,-22,-16,-9,-3,2,6,6,4,1,1,-3,-4,-2,2,7,14,20,26,29,30,28,24,24,21,20,21,25,31,37,44,49,50,50,80];
      | B=[-41.5,-41.5,-63,-20,-63,-20,-63,-20,-41.5,-41.5,-41.5,-34,-26,-21,-20,-22,-28,-37,-47,-57,-63,-63,-54,-44,-34,-26,-21,-20,-22,-28,-37,-47,-57,-63,-63,-54,-44,-34,-26,-21,-20,-22,-28,-37,-47,-57,-63,-63,-54,-44,-34,-26,-21,-20,-22,-28,-37,-41.50,-41.5];
      | plot(A,B);
      | color('black');
      | port_label('LConn', 1, '+')
  86-87 6 : powerlib/Elements/Distributed Parameters Line  Phases=3  Frequency=60  Resistance=R_3  Inductance=L_3  Capacitance=C_3  Length=450*ft2km  x1=[443.88055636918 4247.33488875513 4244.07411041575;376.991118430775 376.991118430775 376.991118430775;-0.417839934887122 0.204452776261364 1.77731617048277]  x2=[443.950645816378 4249.5345875562 4245.8142950916;376.991118430775 376.991118430775 376.991118430775;-0.417953124401402 0.204226490679352 1.77708902793441]  x3=[0.668937841998397 38.9561304156457 40.0687358505382;376.991118430775 376.991118430775 376.991118430775;-1.21872353857018 -1.03942100071866 0.61120852213868]  x4=[0.849863109307604 38.9591215667288 40.1169387971906;376.991118430775 376.991118430775 376.991118430775;0.182472695186911 1.44769825372052 2.94022555594397]  x5=5.64367487766549e-07  V1=ones(3,3)  V2=ones(3,3)  I1=ones(3,3)  I2=ones(3,3)  nHarmo=1  Measurements=None
      settings: SourceProductName=Simscape Electrical
  87 : powerlib/Measurements/Three-Phase V-I Measurement  VoltageMeasurement=phase-to-ground  SetLabelV=on  LabelV=V87  Vpu=off  VpuLL=off  CurrentMeasurement=no  SetLabelI=on  LabelI=I65  Ipu=off  Pbase=100e6  Vbase=24900  OutputType=Complex  PhasorSimulation=on  PSBequivalent=0
      settings: SourceProductName=Simscape Electrical
  87 Y PQ : Subsystem  mask(Single Phase ZIP Load){Vnom=1.0*2401.78, fnom=60, Pnom=40e3*a, Qnom=20e3*a, LoadType=constant P, Vlim=0.7}
      mask prompts: Vnom "Nominal Voltage Vn (Vrms)"; fnom "Nominal Frequency fn (Hz)"; Pnom "Nominal Active power (W)"; Qnom "Nominal Reactive power (VAR)"; LoadType "Load Type"; Vlim "Minimum voltage (pu)"
      mask help:
      | Notes:
      | Single Phase ZIP load model which gets converted to constant Z type if the voltage becomes lower than the Minimum Voltage.
      mask TypeOptions LoadType: Constant Z | constant I | constant P
      mask DialogControl ParameterTabVar0 Prompt: Parameters
      mask DialogControl ParameterTabVar1 Prompt: Type
      mask Display:
      | color('red');
      | A=[-210,-180,-170,-160,-147,-140,-130,-120,-110,-80,-50,-49,-45,-39,-33,-26,-21,-18,-17,-19,-22,-22,-26,-27,-25,-22,-16,-9,-3,2,6,6,4,1,1,-3,-4,-2,2,7,14,20,26,29,30,28,24,24,21,20,21,25,31,37,44,49,50,50,80];
      | B=[-41.5,-41.5,-63,-20,-63,-20,-63,-20,-41.5,-41.5,-41.5,-34,-26,-21,-20,-22,-28,-37,-47,-57,-63,-63,-54,-44,-34,-26,-21,-20,-22,-28,-37,-47,-57,-63,-63,-54,-44,-34,-26,-21,-20,-22,-28,-37,-47,-57,-63,-63,-54,-44,-34,-26,-21,-20,-22,-28,-37,-41.50,-41.5];
      | plot(A,B);
      | color('black');
      | port_label('LConn', 1, '+')
  87-88 9 : powerlib/Elements/Distributed Parameters Line  Phases=1  Frequency=60  Resistance=R_9(1,1)  Inductance=L_9(1,1)  Capacitance=C_9(1,1)  Length=175*ft2km  x1=[3471.63078949902;376.991118430775;-0.0114643872396365]  x2=[3472.97482776458;376.991118430775;-0.0118464386029066]  x3=[30.7628937598647;376.991118430775;-1.37460064138147]  x4=[30.7667057027914;376.991118430775;1.35062140080819]  x5=2.16957196133287e-07  V1=[2.049e+04;377;-2.115]  V2=[2.048e+04;377;-2.115]  I1=[33.62;377;-2.106]  I2=[35.2;377;-2.126]  nHarmo=1  Measurements=None
      settings: SourceProductName=Simscape Electrical
  87-89 6 : powerlib/Elements/Distributed Parameters Line  Phases=3  Frequency=60  Resistance=R_6  Inductance=L_6  Capacitance=C_6  Length=250*ft2km  x1=[446.696793205933 4251.98967952789 4243.32361851028;376.991118430775 376.991118430775 376.991118430775;-1.70866887514147 2.39229582412716 -2.32213671602025]  x2=[446.319152831084 4252.45940668633 4244.33282240905;376.991118430775 376.991118430775 376.991118430775;-1.71238286832956 2.39214212194937 -2.32211697119796]  x3=[16.9729218661877 24.6187204677312 35.6918346381766;376.991118430775 376.991118430775 376.991118430775;1.59405219836339 0.999752717172147 -3.08467723999576]  x4=[18.1321037572291 36.5579826261293 24.6662143427232;376.991118430775 376.991118430775 376.991118430775;-1.55804827623546 3.1166288731389 -0.719283879211711]  x5=3.13537493203638e-07  V1=ones(3,3)  V2=ones(3,3)  I1=ones(3,3)  I2=ones(3,3)  nHarmo=1  Measurements=None
      settings: SourceProductName=Simscape Electrical
  88 : Subsystem
  88 Y CAP : powerlib/Elements/Series RLC Load  LConnTagsString=a  RConnTagsString=__new0  NominalVoltage=1.0*2401.78  NominalFrequency=60  ActivePower=0  InductivePower=0  CapacitivePower=50e3*a  Setx0=off  InitialVoltage=0  SetiL0=off  InitialCurrent=0  Measurements=None  LoadType=constant PQ
      settings: SourceProductName=Simscape Electrical
  88 Y PQ : Subsystem  mask(Single Phase ZIP Load){Vnom=1.0*2401.78, fnom=60, Pnom=40e3*a, Qnom=20e3*a, LoadType=constant P, Vlim=0.7}
      mask prompts: Vnom "Nominal Voltage Vn (Vrms)"; fnom "Nominal Frequency fn (Hz)"; Pnom "Nominal Active power (W)"; Qnom "Nominal Reactive power (VAR)"; LoadType "Load Type"; Vlim "Minimum voltage (pu)"
      mask help:
      | Notes:
      | Single Phase ZIP load model which gets converted to constant Z type if the voltage becomes lower than the Minimum Voltage.
      mask TypeOptions LoadType: Constant Z | constant I | constant P
      mask DialogControl ParameterTabVar0 Prompt: Parameters
      mask DialogControl ParameterTabVar1 Prompt: Type
      mask Display:
      | color('red');
      | A=[-210,-180,-170,-160,-147,-140,-130,-120,-110,-80,-50,-49,-45,-39,-33,-26,-21,-18,-17,-19,-22,-22,-26,-27,-25,-22,-16,-9,-3,2,6,6,4,1,1,-3,-4,-2,2,7,14,20,26,29,30,28,24,24,21,20,21,25,31,37,44,49,50,50,80];
      | B=[-41.5,-41.5,-63,-20,-63,-20,-63,-20,-41.5,-41.5,-41.5,-34,-26,-21,-20,-22,-28,-37,-47,-57,-63,-63,-54,-44,-34,-26,-21,-20,-22,-28,-37,-47,-57,-63,-63,-54,-44,-34,-26,-21,-20,-22,-28,-37,-47,-57,-63,-63,-54,-44,-34,-26,-21,-20,-22,-28,-37,-41.50,-41.5];
      | plot(A,B);
      | color('black');
      | port_label('LConn', 1, '+')
  89 : powerlib/Measurements/Three-Phase V-I Measurement  VoltageMeasurement=phase-to-ground  SetLabelV=on  LabelV=V89  Vpu=off  VpuLL=off  CurrentMeasurement=no  SetLabelI=on  LabelI=I65  Ipu=off  Pbase=100e6  Vbase=24900  OutputType=Complex  PhasorSimulation=on  PSBequivalent=0
      settings: SourceProductName=Simscape Electrical
  89-90 10 : powerlib/Elements/Distributed Parameters Line  Phases=1  Frequency=60  Resistance=R_10(2,2)  Inductance=L_10(2,2)  Capacitance=C_10(2,2)  Length=225*ft2km  x1=[3468.32033788323;376.991118430775;-2.10640475425775]  x2=[3470.04684143222;376.991118430775;-2.10689601869891]  x3=[30.7359181752822;376.991118430775;2.81351521758528]  x4=[30.7404050902913;376.991118430775;-0.74442700932166]  x5=2.78944966457084e-07  V1=[2.049e+04;377;-2.115]  V2=[2.048e+04;377;-2.115]  I1=[33.62;377;-2.106]  I2=[35.2;377;-2.126]  nHarmo=1  Measurements=None
      settings: SourceProductName=Simscape Electrical
  89-91 6 : powerlib/Elements/Distributed Parameters Line  Phases=3  Frequency=60  Resistance=R_6  Inductance=L_6  Capacitance=C_6  Length=225*ft2km  x1=[446.319152831084 4252.45940668633 4244.33282240905;376.991118430775 376.991118430775 376.991118430775;-1.71237104824454 2.39215192889734 -2.32210720690629]  x2=[444.874787313719 4252.91460611842 4244.52373103371;376.991118430775 376.991118430775 376.991118430775;-1.71328354154684 2.39203906725925 -2.32205574407447]  x3=[16.8552697039191 24.8287894670264 21.1831423457523;376.991118430775 376.991118430775 376.991118430775;0.486306760165325 1.16893556360892 -2.4494153155459]  x4=[17.5694177617675 32.9738910819185 4.82774348265843;376.991118430775 376.991118430775 376.991118430775;-2.60132509891296 -3.10457238754497 -1.7313384371018]  x5=2.82183743883275e-07  V1=ones(3,3)  V2=ones(3,3)  I1=ones(3,3)  I2=ones(3,3)  nHarmo=1  Measurements=None
      settings: SourceProductName=Simscape Electrical
  9 : Subsystem
  9 Y PQ : Subsystem  mask(Single Phase ZIP Load){Vnom=1.0*2401.78, fnom=60, Pnom=40e3*a, Qnom=20e3*a, LoadType=constant P, Vlim=0.7}
      mask prompts: Vnom "Nominal Voltage Vn (Vrms)"; fnom "Nominal Frequency fn (Hz)"; Pnom "Nominal Active power (W)"; Qnom "Nominal Reactive power (VAR)"; LoadType "Load Type"; Vlim "Minimum voltage (pu)"
      mask help:
      | Notes:
      | Single Phase ZIP load model which gets converted to constant Z type if the voltage becomes lower than the Minimum Voltage.
      mask TypeOptions LoadType: Constant Z | constant I | constant P
      mask DialogControl ParameterTabVar0 Prompt: Parameters
      mask DialogControl ParameterTabVar1 Prompt: Type
      mask Display:
      | color('red');
      | A=[-210,-180,-170,-160,-147,-140,-130,-120,-110,-80,-50,-49,-45,-39,-33,-26,-21,-18,-17,-19,-22,-22,-26,-27,-25,-22,-16,-9,-3,2,6,6,4,1,1,-3,-4,-2,2,7,14,20,26,29,30,28,24,24,21,20,21,25,31,37,44,49,50,50,80];
      | B=[-41.5,-41.5,-63,-20,-63,-20,-63,-20,-41.5,-41.5,-41.5,-34,-26,-21,-20,-22,-28,-37,-47,-57,-63,-63,-54,-44,-34,-26,-21,-20,-22,-28,-37,-47,-57,-63,-63,-54,-44,-34,-26,-21,-20,-22,-28,-37,-47,-57,-63,-63,-54,-44,-34,-26,-21,-20,-22,-28,-37,-41.50,-41.5];
      | plot(A,B);
      | color('black');
      | port_label('LConn', 1, '+')
  9-14 9 : powerlib/Elements/Distributed Parameters Line  Phases=1  Frequency=60  Resistance=R_9(1,1)  Inductance=L_9(1,1)  Capacitance=C_9(1,1)  Length=425*ft2km  x1=[3412.46894024718;376.991118430775;-0.00336744664739336]  x2=[3412.46807066232;376.991118430775;-0.0033678372870635]  x3=[6.23826866467113;376.991118430775;-0.00380049994556681]  x4=[6.25873946062357;376.991118430775;-0.00313451976245101]  x5=5.26896047752269e-07  V1=[2.049e+04;377;-2.115]  V2=[2.048e+04;377;-2.115]  I1=[33.62;377;-2.106]  I2=[35.2;377;-2.126]  nHarmo=1  Measurements=None
      settings: SourceProductName=Simscape Electrical
  90 : Subsystem
  90 Y CAP : powerlib/Elements/Series RLC Load  LConnTagsString=a  RConnTagsString=__new0  NominalVoltage=1.0*2401.78  NominalFrequency=60  ActivePower=0  InductivePower=0  CapacitivePower=50e3*a  Setx0=off  InitialVoltage=0  SetiL0=off  InitialCurrent=0  Measurements=None  LoadType=constant PQ
      settings: SourceProductName=Simscape Electrical
  90 Y I : Subsystem  mask(Single Phase ZIP Load){Vnom=1.0*2401.78, fnom=60, Pnom=40e3*a, Qnom=20e3*a, LoadType=constant I, Vlim=0.7}
      mask prompts: Vnom "Nominal Voltage Vn (Vrms)"; fnom "Nominal Frequency fn (Hz)"; Pnom "Nominal Active power (W)"; Qnom "Nominal Reactive power (VAR)"; LoadType "Load Type"; Vlim "Minimum voltage (pu)"
      mask help:
      | Notes:
      | Single Phase ZIP load model which gets converted to constant Z type if the voltage becomes lower than the Minimum Voltage.
      mask TypeOptions LoadType: Constant Z | constant I | constant P
      mask DialogControl ParameterTabVar0 Prompt: Parameters
      mask DialogControl ParameterTabVar1 Prompt: Type
      mask Display:
      | color('red');
      | A=[-210,-180,-170,-160,-147,-140,-130,-120,-110,-80,-50,-49,-45,-39,-33,-26,-21,-18,-17,-19,-22,-22,-26,-27,-25,-22,-16,-9,-3,2,6,6,4,1,1,-3,-4,-2,2,7,14,20,26,29,30,28,24,24,21,20,21,25,31,37,44,49,50,50,80];
      | B=[-41.5,-41.5,-63,-20,-63,-20,-63,-20,-41.5,-41.5,-41.5,-34,-26,-21,-20,-22,-28,-37,-47,-57,-63,-63,-54,-44,-34,-26,-21,-20,-22,-28,-37,-47,-57,-63,-63,-54,-44,-34,-26,-21,-20,-22,-28,-37,-47,-57,-63,-63,-54,-44,-34,-26,-21,-20,-22,-28,-37,-41.50,-41.5];
      | plot(A,B);
      | color('black');
      | port_label('LConn', 1, '+')
  91 : powerlib/Measurements/Three-Phase V-I Measurement  VoltageMeasurement=phase-to-ground  SetLabelV=on  LabelV=V91  Vpu=off  VpuLL=off  CurrentMeasurement=no  SetLabelI=on  LabelI=I65  Ipu=off  Pbase=100e6  Vbase=24900  OutputType=Complex  PhasorSimulation=on  PSBequivalent=0
      settings: SourceProductName=Simscape Electrical
  91-92 11 : powerlib/Elements/Distributed Parameters Line  Phases=1  Frequency=60  Resistance=R_11(3,3)  Inductance=L_11(3,3)  Capacitance=C_11(3,3)  Length=300*ft2km  x1=[3472.65933187463;376.991118430775;2.08525434621725]  x2=[3474.96442103075;376.991118430775;2.08459921584575]  x3=[30.7779132541919;376.991118430775;0.721795335767785]  x4=[30.7834252989769;376.991118430775;-2.83611533397464]  x5=3.71926621942778e-07  V1=[2.049e+04;377;-2.115]  V2=[2.048e+04;377;-2.115]  I1=[33.62;377;-2.106]  I2=[35.2;377;-2.126]  nHarmo=1  Measurements=None
      settings: SourceProductName=Simscape Electrical
  91-93 6 : powerlib/Elements/Distributed Parameters Line  Phases=3  Frequency=60  Resistance=R_6  Inductance=L_6  Capacitance=C_6  Length=225*ft2km  x1=[444.874787313719 4252.91460611842 4244.52373103372;376.991118430775 376.991118430775 376.991118430775;-1.71328354154684 2.39203906725925 -2.32205574407447]  x2=[444.874751146581 4252.91466572258 4244.52371248732;376.991118430775 376.991118430775 376.991118430775;-1.71328418340535 2.39203904898463 -2.32205579860416]  x3=[0.581537434785637 15.8736654826457 12.5041420783171;376.991118430775 376.991118430775 376.991118430775;-1.7147715889969 2.39178560621416 -2.3222857017605]  x4=[0.587924047909405 15.8765715285433 12.5176361129502;376.991118430775 376.991118430775 376.991118430775;-1.7119181011998 2.39220420810835 -2.32191392088563]  x5=2.82183743883275e-07  V1=ones(3,3)  V2=ones(3,3)  I1=ones(3,3)  I2=ones(3,3)  nHarmo=1  Measurements=None
      settings: SourceProductName=Simscape Electrical
  92 : Subsystem
  92 Y CAP : powerlib/Elements/Series RLC Load  LConnTagsString=a  RConnTagsString=__new0  NominalVoltage=1.0*2401.78  NominalFrequency=60  ActivePower=0  InductivePower=0  CapacitivePower=50e3*a  Setx0=off  InitialVoltage=0  SetiL0=off  InitialCurrent=0  Measurements=None  LoadType=constant PQ
      settings: SourceProductName=Simscape Electrical
  92 Y PQ : Subsystem  mask(Single Phase ZIP Load){Vnom=1.0*2401.78, fnom=60, Pnom=40e3*a, Qnom=20e3*a, LoadType=constant P, Vlim=0.7}
      mask prompts: Vnom "Nominal Voltage Vn (Vrms)"; fnom "Nominal Frequency fn (Hz)"; Pnom "Nominal Active power (W)"; Qnom "Nominal Reactive power (VAR)"; LoadType "Load Type"; Vlim "Minimum voltage (pu)"
      mask help:
      | Notes:
      | Single Phase ZIP load model which gets converted to constant Z type if the voltage becomes lower than the Minimum Voltage.
      mask TypeOptions LoadType: Constant Z | constant I | constant P
      mask DialogControl ParameterTabVar0 Prompt: Parameters
      mask DialogControl ParameterTabVar1 Prompt: Type
      mask Display:
      | color('red');
      | A=[-210,-180,-170,-160,-147,-140,-130,-120,-110,-80,-50,-49,-45,-39,-33,-26,-21,-18,-17,-19,-22,-22,-26,-27,-25,-22,-16,-9,-3,2,6,6,4,1,1,-3,-4,-2,2,7,14,20,26,29,30,28,24,24,21,20,21,25,31,37,44,49,50,50,80];
      | B=[-41.5,-41.5,-63,-20,-63,-20,-63,-20,-41.5,-41.5,-41.5,-34,-26,-21,-20,-22,-28,-37,-47,-57,-63,-63,-54,-44,-34,-26,-21,-20,-22,-28,-37,-47,-57,-63,-63,-54,-44,-34,-26,-21,-20,-22,-28,-37,-47,-57,-63,-63,-54,-44,-34,-26,-21,-20,-22,-28,-37,-41.50,-41.5];
      | plot(A,B);
      | color('black');
      | port_label('LConn', 1, '+')
  93 : powerlib/Measurements/Three-Phase V-I Measurement  VoltageMeasurement=phase-to-ground  SetLabelV=on  LabelV=V93  Vpu=off  VpuLL=off  CurrentMeasurement=no  SetLabelI=on  LabelI=I65  Ipu=off  Pbase=100e6  Vbase=24900  OutputType=Complex  PhasorSimulation=on  PSBequivalent=0
      settings: SourceProductName=Simscape Electrical
  93-94 9 : powerlib/Elements/Distributed Parameters Line  Phases=1  Frequency=60  Resistance=R_9(1,1)  Inductance=L_9(1,1)  Capacitance=C_9(1,1)  Length=275*ft2km  x1=[3470.88215405092;376.991118430775;-0.0112135375417357]  x2=[3470.88193859184;376.991118430775;-0.0112136163902688]  x3=[6.35228243333851;376.991118430775;-0.0113397926158146]  x4=[6.35930402098953;376.991118430775;-0.0112159624041424]  x5=3.4093273678088e-07  V1=[2.049e+04;377;-2.115]  V2=[2.048e+04;377;-2.115]  I1=[33.62;377;-2.106]  I2=[35.2;377;-2.126]  nHarmo=1  Measurements=None
      settings: SourceProductName=Simscape Electrical
  93-95 6 : powerlib/Elements/Distributed Parameters Line  Phases=3  Frequency=60  Resistance=R_6  Inductance=L_6  Capacitance=C_6  Length=300*ft2km  x1=[444.874751146581 4252.91466572258 4244.52371248732;376.991118430775 376.991118430775 376.991118430775;-1.71331964366042 2.3920096281407 -2.32208509147917]  x2=[444.874451027264 4252.91466105594 4244.52371663196;376.991118430775 376.991118430775 376.991118430775;-1.71332047833812 2.39200962598739 -2.3220851473293]  x3=[0.580800127612022 15.8746396764565 12.5057998113134;376.991118430775 376.991118430775 376.991118430775;-1.7113137852491 2.39195019057326 -2.32232564151661]  x4=[0.588649736071026 15.8752102027081 12.5157381720135;376.991118430775 376.991118430775 376.991118430775;-1.71544048046698 2.39195137824748 -2.32196191476106]  x5=3.76244991844366e-07  V1=ones(3,3)  V2=ones(3,3)  I1=ones(3,3)  I2=ones(3,3)  nHarmo=1  Measurements=None
      settings: SourceProductName=Simscape Electrical
  94 : Subsystem
  94 Y PQ : Subsystem  mask(Single Phase ZIP Load){Vnom=1.0*2401.78, fnom=60, Pnom=40e3*a, Qnom=20e3*a, LoadType=constant P, Vlim=0.7}
      mask prompts: Vnom "Nominal Voltage Vn (Vrms)"; fnom "Nominal Frequency fn (Hz)"; Pnom "Nominal Active power (W)"; Qnom "Nominal Reactive power (VAR)"; LoadType "Load Type"; Vlim "Minimum voltage (pu)"
      mask help:
      | Notes:
      | Single Phase ZIP load model which gets converted to constant Z type if the voltage becomes lower than the Minimum Voltage.
      mask TypeOptions LoadType: Constant Z | constant I | constant P
      mask DialogControl ParameterTabVar0 Prompt: Parameters
      mask DialogControl ParameterTabVar1 Prompt: Type
      mask Display:
      | color('red');
      | A=[-210,-180,-170,-160,-147,-140,-130,-120,-110,-80,-50,-49,-45,-39,-33,-26,-21,-18,-17,-19,-22,-22,-26,-27,-25,-22,-16,-9,-3,2,6,6,4,1,1,-3,-4,-2,2,7,14,20,26,29,30,28,24,24,21,20,21,25,31,37,44,49,50,50,80];
      | B=[-41.5,-41.5,-63,-20,-63,-20,-63,-20,-41.5,-41.5,-41.5,-34,-26,-21,-20,-22,-28,-37,-47,-57,-63,-63,-54,-44,-34,-26,-21,-20,-22,-28,-37,-47,-57,-63,-63,-54,-44,-34,-26,-21,-20,-22,-28,-37,-47,-57,-63,-63,-54,-44,-34,-26,-21,-20,-22,-28,-37,-41.50,-41.5];
      | plot(A,B);
      | color('black');
      | port_label('LConn', 1, '+')
  95 : powerlib/Measurements/Three-Phase V-I Measurement  VoltageMeasurement=phase-to-ground  SetLabelV=on  LabelV=V95  Vpu=off  VpuLL=off  CurrentMeasurement=no  SetLabelI=on  LabelI=I65  Ipu=off  Pbase=100e6  Vbase=24900  OutputType=Complex  PhasorSimulation=on  PSBequivalent=0
      settings: SourceProductName=Simscape Electrical
  95 Y PQ : Subsystem  mask(Single Phase ZIP Load){Vnom=1.0*2401.78, fnom=60, Pnom=20e3*a, Qnom=10e3*a, LoadType=constant P, Vlim=0.7}
      mask prompts: Vnom "Nominal Voltage Vn (Vrms)"; fnom "Nominal Frequency fn (Hz)"; Pnom "Nominal Active power (W)"; Qnom "Nominal Reactive power (VAR)"; LoadType "Load Type"; Vlim "Minimum voltage (pu)"
      mask help:
      | Notes:
      | Single Phase ZIP load model which gets converted to constant Z type if the voltage becomes lower than the Minimum Voltage.
      mask TypeOptions LoadType: Constant Z | constant I | constant P
      mask DialogControl ParameterTabVar0 Prompt: Parameters
      mask DialogControl ParameterTabVar1 Prompt: Type
      mask Display:
      | color('red');
      | A=[-210,-180,-170,-160,-147,-140,-130,-120,-110,-80,-50,-49,-45,-39,-33,-26,-21,-18,-17,-19,-22,-22,-26,-27,-25,-22,-16,-9,-3,2,6,6,4,1,1,-3,-4,-2,2,7,14,20,26,29,30,28,24,24,21,20,21,25,31,37,44,49,50,50,80];
      | B=[-41.5,-41.5,-63,-20,-63,-20,-63,-20,-41.5,-41.5,-41.5,-34,-26,-21,-20,-22,-28,-37,-47,-57,-63,-63,-54,-44,-34,-26,-21,-20,-22,-28,-37,-47,-57,-63,-63,-54,-44,-34,-26,-21,-20,-22,-28,-37,-47,-57,-63,-63,-54,-44,-34,-26,-21,-20,-22,-28,-37,-41.50,-41.5];
      | plot(A,B);
      | color('black');
      | port_label('LConn', 1, '+')
  95-96 10 : powerlib/Elements/Distributed Parameters Line  Phases=1  Frequency=60  Resistance=R_10(2,2)  Inductance=L_10(2,2)  Capacitance=C_10(2,2)  Length=200*ft2km  x1=[3467.87624270705;376.991118430775;-2.10650093307156]  x2=[3467.87608325492;376.991118430775;-2.10650098842285]  x3=[6.34698604279021;376.991118430775;-2.10659446181917]  x4=[6.3539211546601;376.991118430775;-2.10650098822515]  x5=2.47951081295186e-07  V1=[2.049e+04;377;-2.115]  V2=[2.048e+04;377;-2.115]  I1=[33.62;377;-2.106]  I2=[35.2;377;-2.126]  nHarmo=1  Measurements=None
      settings: SourceProductName=Simscape Electrical
  96 : Subsystem
  96 Y PQ : Subsystem  mask(Single Phase ZIP Load){Vnom=1.0*2401.78, fnom=60, Pnom=20e3*a, Qnom=10e3*a, LoadType=constant P, Vlim=0.7}
      mask prompts: Vnom "Nominal Voltage Vn (Vrms)"; fnom "Nominal Frequency fn (Hz)"; Pnom "Nominal Active power (W)"; Qnom "Nominal Reactive power (VAR)"; LoadType "Load Type"; Vlim "Minimum voltage (pu)"
      mask help:
      | Notes:
      | Single Phase ZIP load model which gets converted to constant Z type if the voltage becomes lower than the Minimum Voltage.
      mask TypeOptions LoadType: Constant Z | constant I | constant P
      mask DialogControl ParameterTabVar0 Prompt: Parameters
      mask DialogControl ParameterTabVar1 Prompt: Type
      mask Display:
      | color('red');
      | A=[-210,-180,-170,-160,-147,-140,-130,-120,-110,-80,-50,-49,-45,-39,-33,-26,-21,-18,-17,-19,-22,-22,-26,-27,-25,-22,-16,-9,-3,2,6,6,4,1,1,-3,-4,-2,2,7,14,20,26,29,30,28,24,24,21,20,21,25,31,37,44,49,50,50,80];
      | B=[-41.5,-41.5,-63,-20,-63,-20,-63,-20,-41.5,-41.5,-41.5,-34,-26,-21,-20,-22,-28,-37,-47,-57,-63,-63,-54,-44,-34,-26,-21,-20,-22,-28,-37,-47,-57,-63,-63,-54,-44,-34,-26,-21,-20,-22,-28,-37,-47,-57,-63,-63,-54,-44,-34,-26,-21,-20,-22,-28,-37,-41.50,-41.5];
      | plot(A,B);
      | color('black');
      | port_label('LConn', 1, '+')
  97 : powerlib/Measurements/Three-Phase V-I Measurement  VoltageMeasurement=phase-to-ground  SetLabelV=on  LabelV=V97  Vpu=off  VpuLL=off  CurrentMeasurement=no  SetLabelI=on  LabelI=I65  Ipu=off  Pbase=100e6  Vbase=24900  OutputType=Complex  PhasorSimulation=on  PSBequivalent=0
      settings: SourceProductName=Simscape Electrical
  97-1 : powerlib/Elements/Three-Phase Breaker  InitialState=closed  SwitchA=off  SwitchB=off  SwitchC=off  SwitchTimes="[1/60  5/60]"  External=off  BreakerResistance=1e-6  SnubberResistance=1e6  SnubberCapacitance=inf  Measurements=None
      settings: SourceProductName=Simscape Electrical
  97-98 3 : powerlib/Elements/Distributed Parameters Line  Phases=3  Frequency=60  Resistance=R_3  Inductance=L_3  Capacitance=C_3  Length=275*ft2km  x1=[443.373227084636 4232.2593632206 4232.16270175339;376.991118430775 376.991118430775 376.991118430775;-0.41697765188343 0.206083281224702 1.77895325774172]  x2=[443.373272039753 4232.25961324745 4232.16295426825;376.991118430775 376.991118430775 376.991118430775;-0.416977707600537 0.206083211990193 1.77895318709348]  x3=[0.582694580500708 12.4704277678166 15.7932985676371;376.991118430775 376.991118430775 376.991118430775;-0.417862558528328 0.205330967171377 1.77819809886902]  x4=[0.582810708769499 12.4788978848887 15.8017658861111;376.991118430775 376.991118430775 376.991118430775;-0.416222986962726 0.206727643409429 1.77960009220308]  x5=3.44891242524002e-07  V1=ones(3,3)  V2=ones(3,3)  I1=ones(3,3)  I2=ones(3,3)  nHarmo=1  Measurements=None
      settings: SourceProductName=Simscape Electrical
  98 : powerlib/Measurements/Three-Phase V-I Measurement  VoltageMeasurement=phase-to-ground  SetLabelV=on  LabelV=V98  Vpu=off  VpuLL=off  CurrentMeasurement=no  SetLabelI=on  LabelI=I65  Ipu=off  Pbase=100e6  Vbase=24900  OutputType=Complex  PhasorSimulation=on  PSBequivalent=0
      settings: SourceProductName=Simscape Electrical
  98 Y PQ : Subsystem  mask(Single Phase ZIP Load){Vnom=1.0*2401.78, fnom=60, Pnom=40e3*a, Qnom=20e3*a, LoadType=constant P, Vlim=0.7}
      mask prompts: Vnom "Nominal Voltage Vn (Vrms)"; fnom "Nominal Frequency fn (Hz)"; Pnom "Nominal Active power (W)"; Qnom "Nominal Reactive power (VAR)"; LoadType "Load Type"; Vlim "Minimum voltage (pu)"
      mask help:
      | Notes:
      | Single Phase ZIP load model which gets converted to constant Z type if the voltage becomes lower than the Minimum Voltage.
      mask TypeOptions LoadType: Constant Z | constant I | constant P
      mask DialogControl ParameterTabVar0 Prompt: Parameters
      mask DialogControl ParameterTabVar1 Prompt: Type
      mask Display:
      | color('red');
      | A=[-210,-180,-170,-160,-147,-140,-130,-120,-110,-80,-50,-49,-45,-39,-33,-26,-21,-18,-17,-19,-22,-22,-26,-27,-25,-22,-16,-9,-3,2,6,6,4,1,1,-3,-4,-2,2,7,14,20,26,29,30,28,24,24,21,20,21,25,31,37,44,49,50,50,80];
      | B=[-41.5,-41.5,-63,-20,-63,-20,-63,-20,-41.5,-41.5,-41.5,-34,-26,-21,-20,-22,-28,-37,-47,-57,-63,-63,-54,-44,-34,-26,-21,-20,-22,-28,-37,-47,-57,-63,-63,-54,-44,-34,-26,-21,-20,-22,-28,-37,-47,-57,-63,-63,-54,-44,-34,-26,-21,-20,-22,-28,-37,-41.50,-41.5];
      | plot(A,B);
      | color('black');
      | port_label('LConn', 1, '+')
  98-99 3 : powerlib/Elements/Distributed Parameters Line  Phases=3  Frequency=60  Resistance=R_3  Inductance=L_3  Capacitance=C_3  Length=550*ft2km  x1=[443.373272039753 4232.25961324745 4232.16295426825;376.991118430775 376.991118430775 376.991118430775;-0.417107728535793 0.20597580478183 1.77884531066574]  x2=[443.373328294253 4232.2600877318 4232.16328788012;376.991118430775 376.991118430775 376.991118430775;-0.417106836593731 0.205975720733782 1.77884519364367]  x3=[0.584549762148562 12.4725140589008 15.7927004707388;376.991118430775 376.991118430775 376.991118430775;-0.416474705893538 0.205286498973157 1.77822774301059]  x4=[0.580910022099564 12.4759339311809 15.8009518283575;376.991118430775 376.991118430775 376.991118430775;-0.418004686004984 0.206450047589944 1.77924673588914]  x5=6.89782485048005e-07  V1=ones(3,3)  V2=ones(3,3)  I1=ones(3,3)  I2=ones(3,3)  nHarmo=1  Measurements=None
      settings: SourceProductName=Simscape Electrical
  99 : powerlib/Measurements/Three-Phase V-I Measurement  VoltageMeasurement=phase-to-ground  SetLabelV=on  LabelV=V99  Vpu=off  VpuLL=off  CurrentMeasurement=no  SetLabelI=on  LabelI=I65  Ipu=off  Pbase=100e6  Vbase=24900  OutputType=Complex  PhasorSimulation=on  PSBequivalent=0
      settings: SourceProductName=Simscape Electrical
  99 Y PQ : Subsystem  mask(Single Phase ZIP Load){Vnom=1.0*2401.78, fnom=60, Pnom=40e3*a, Qnom=20e3*a, LoadType=constant P, Vlim=0.7}
      mask prompts: Vnom "Nominal Voltage Vn (Vrms)"; fnom "Nominal Frequency fn (Hz)"; Pnom "Nominal Active power (W)"; Qnom "Nominal Reactive power (VAR)"; LoadType "Load Type"; Vlim "Minimum voltage (pu)"
      mask help:
      | Notes:
      | Single Phase ZIP load model which gets converted to constant Z type if the voltage becomes lower than the Minimum Voltage.
      mask TypeOptions LoadType: Constant Z | constant I | constant P
      mask DialogControl ParameterTabVar0 Prompt: Parameters
      mask DialogControl ParameterTabVar1 Prompt: Type
      mask Display:
      | color('red');
      | A=[-210,-180,-170,-160,-147,-140,-130,-120,-110,-80,-50,-49,-45,-39,-33,-26,-21,-18,-17,-19,-22,-22,-26,-27,-25,-22,-16,-9,-3,2,6,6,4,1,1,-3,-4,-2,2,7,14,20,26,29,30,28,24,24,21,20,21,25,31,37,44,49,50,50,80];
      | B=[-41.5,-41.5,-63,-20,-63,-20,-63,-20,-41.5,-41.5,-41.5,-34,-26,-21,-20,-22,-28,-37,-47,-57,-63,-63,-54,-44,-34,-26,-21,-20,-22,-28,-37,-47,-57,-63,-63,-54,-44,-34,-26,-21,-20,-22,-28,-37,-47,-57,-63,-63,-54,-44,-34,-26,-21,-20,-22,-28,-37,-41.50,-41.5];
      | plot(A,B);
      | color('black');
      | port_label('LConn', 1, '+')
  99-100 3 : powerlib/Elements/Distributed Parameters Line  Phases=3  Frequency=60  Resistance=R_3  Inductance=L_3  Capacitance=C_3  Length=300*ft2km  x1=[443.373328294253 4232.2600877318 4232.16328788012;376.991118430775 376.991118430775 376.991118430775;-0.416988635743498 0.206073363650476 1.77894326312344]  x2=[443.373552146088 4232.26022753008 4232.1634537403;376.991118430775 376.991118430775 376.991118430775;-0.416988389854877 0.206073345723561 1.77894321545756]  x3=[0.584339351330208 12.4743098706746 15.7947887979546;376.991118430775 376.991118430775 376.991118430775;-0.419519683522342 0.205721911439559 1.7784577210148]  x4=[0.581165449449398 12.474934897556 15.8001465698015;376.991118430775 376.991118430775 376.991118430775;-0.414585748976709 0.206307610263959 1.7793109275976]  x5=3.76244991844366e-07  V1=ones(3,3)  V2=ones(3,3)  I1=ones(3,3)  I2=ones(3,3)  nHarmo=1  Measurements=None
      settings: SourceProductName=Simscape Electrical
  Ground{,1..81} (82 alike) : powerlib/Elements/Ground  LConnTagsString=a
      settings: SourceProductName=Simscape Electrical
  Load Flow Bus10 : powerlib/Measurements/Load Flow Bus  LConnTagsString=a|b|c  Phases=ABC  Connectors=on one side  ID=251  Vbase=4160/sqrt(3)  Vref=[1.0 1.0 1.0]  Vangle=[0 -120 120]  VLF=1  VLFb=1  VLFc=1  angleLF=0  angleLFb=0  angleLFc=0
      settings: SourceProductName=Simscape Electrical
  Load Flow Bus106 : powerlib/Measurements/Load Flow Bus  LConnTagsString=a|b|c  RConnTagsString=a|b|c  Phases=ABC  Connectors=on both sides  ID=450  Vbase=4160/sqrt(3)  Vref=[1.0 1.0 1.0]  Vangle=[0 -120 120]  VLF=1  VLFb=1  VLFc=1  angleLF=0  angleLFb=0  angleLFc=0
      settings: SourceProductName=Simscape Electrical
  Load Flow Bus107 : powerlib/Measurements/Load Flow Bus  LConnTagsString=a|b|c  Phases=ABC  Connectors=on one side  ID=451  Vbase=4160/sqrt(3)  Vref=[1.0 1.0 1.0]  Vangle=[0 -120 120]  VLF=1  VLFb=1  VLFc=1  angleLF=0  angleLFb=0  angleLFc=0
      settings: SourceProductName=Simscape Electrical
  Load Flow Bus117 : powerlib/Measurements/Load Flow Bus  LConnTagsString=a|b|c  Phases=ABC  Connectors=on one side  ID=79  Vbase=4160/sqrt(3)  Vref=[1.0 1.0 1.0]  Vangle=[0 -120 120]  VLF=1  VLFb=1  VLFc=1  angleLF=0  angleLFb=0  angleLFc=0
      settings: SourceProductName=Simscape Electrical
  Load Flow Bus128 : powerlib/Measurements/Load Flow Bus  LConnTagsString=a|b|c  Phases=ABC  Connectors=on one side  ID=66  Vbase=4160/sqrt(3)  Vref=[1.0 1.0 1.0]  Vangle=[0 -120 120]  VLF=1  VLFb=1  VLFc=1  angleLF=0  angleLFb=0  angleLFc=0
      settings: SourceProductName=Simscape Electrical
  Load Flow Bus2 : powerlib/Measurements/Load Flow Bus  LConnTagsString=a|b|c  RConnTagsString=a|b|c  Phases=ABC  Connectors=on both sides  ID=36  Vbase=4160/sqrt(3)  Vref=[1.0 1.0]  Vangle=[0 -120]  VLF=1  VLFb=1  VLFc=1  angleLF=0  angleLFb=0  angleLFc=0
      settings: SourceProductName=Simscape Electrical
  Load Flow Bus44 : powerlib/Measurements/Load Flow Bus  LConnTagsString=a|b|c  RConnTagsString=a|b|c  Phases=ABC  Connectors=on both sides  ID=300  Vbase=4160/sqrt(3)  Vref=[1.0 1.0 1.0]  Vangle=[0 -120 120]  VLF=1  VLFb=1  VLFc=1  angleLF=0  angleLFb=0  angleLFc=0
      settings: SourceProductName=Simscape Electrical
  Load Flow Bus45 : powerlib/Measurements/Load Flow Bus  LConnTagsString=a|b|c  Phases=ABC  Connectors=on one side  ID=350  Vbase=4160/sqrt(3)  Vref=[1.0 1.0 1.0]  Vangle=[0 -120 120]  VLF=1  VLFb=1  VLFc=1  angleLF=0  angleLFb=0  angleLFc=0
      settings: SourceProductName=Simscape Electrical
  Load Flow Bus55 : powerlib/Measurements/Load Flow Bus  LConnTagsString=a|b  RConnTagsString=a|b  Phases=AB  Connectors=on both sides  ID=36  Vbase=4160/sqrt(3)  Vref=[1.0 1.0]  Vangle=[0 -120]  VLF=1  VLFb=1  VLFc=1  angleLF=0  angleLFb=0  angleLFc=0
      settings: SourceProductName=Simscape Electrical
  Load Flow Bus68 : powerlib/Measurements/Load Flow Bus  LConnTagsString=a|b|c  Phases=ABC  Connectors=on one side  ID=56  Vbase=4160/sqrt(3)  Vref=[1.0 1.0 1.0]  Vangle=[0 -120 120]  VLF=1  VLFb=1  VLFc=1  angleLF=0  angleLFb=0  angleLFc=0
      settings: SourceProductName=Simscape Electrical
  Load Flow Bus77 : powerlib/Measurements/Load Flow Bus  LConnTagsString=a|b|c  RConnTagsString=a|b|c  Phases=ABC  Connectors=on both sides  ID=95  Vbase=4160/sqrt(3)  Vref=[1.0 1.0 1.0]  Vangle=[0 -120 120]  VLF=1  VLFb=1  VLFc=1  angleLF=0  angleLFb=0  angleLFc=0
      settings: SourceProductName=Simscape Electrical
  Load Flow Bus78 : powerlib/Measurements/Load Flow Bus  LConnTagsString=a|b|c  Phases=ABC  Connectors=on one side  ID=195  Vbase=4160/sqrt(3)  Vref=[1.0 1.0 1.0]  Vangle=[0 -120 120]  VLF=1  VLFb=1  VLFc=1  angleLF=0  angleLFb=0  angleLFc=0
      settings: SourceProductName=Simscape Electrical
  Load Flow Bus84 : powerlib/Measurements/Load Flow Bus  LConnTagsString=a|b|c  Phases=ABC  Connectors=on one side  ID=610  Vbase=480/sqrt(3)  Vref=[0.98860 1.0256 1.0052]  Vangle=[-3.51 -122 117.5]  VLF=1  VLFb=1  VLFc=1  angleLF=0  angleLFb=0  angleLFc=0
      settings: SourceProductName=Simscape Electrical
  Measurements : Subsystem
  RG1in : powerlib/Measurements/Three-Phase V-I Measurement  VoltageMeasurement=phase-to-ground  SetLabelV=on  LabelV=RG1in  Vpu=off  VpuLL=off  CurrentMeasurement=no  SetLabelI=on  LabelI=I800  Ipu=off  Pbase=100e6  Vbase=24900  OutputType=Complex  PhasorSimulation=on  PSBequivalent=0
      settings: SourceProductName=Simscape Electrical
  RG1out : powerlib/Measurements/Three-Phase V-I Measurement  VoltageMeasurement=phase-to-ground  SetLabelV=on  LabelV=RG1out  Vpu=off  VpuLL=off  CurrentMeasurement=no  SetLabelI=on  LabelI=I800  Ipu=off  Pbase=100e6  Vbase=24900  OutputType=Complex  PhasorSimulation=on  PSBequivalent=0
      settings: SourceProductName=Simscape Electrical
  RG2in : Subsystem
  RG2out : Subsystem
  RG3in : Subsystem
  RG3out : Subsystem
  RG4in : powerlib/Measurements/Three-Phase V-I Measurement  VoltageMeasurement=phase-to-ground  SetLabelV=on  LabelV=RG4in  Vpu=off  VpuLL=off  CurrentMeasurement=no  SetLabelI=on  LabelI=I800  Ipu=off  Pbase=100e6  Vbase=24900  OutputType=Complex  PhasorSimulation=on  PSBequivalent=0
      settings: SourceProductName=Simscape Electrical
  RG4out : powerlib/Measurements/Three-Phase V-I Measurement  VoltageMeasurement=phase-to-ground  SetLabelV=on  LabelV=RG4out  Vpu=off  VpuLL=off  CurrentMeasurement=no  SetLabelI=on  LabelI=I800  Ipu=off  Pbase=100e6  Vbase=24900  OutputType=Complex  PhasorSimulation=on  PSBequivalent=0
      settings: SourceProductName=Simscape Electrical
  Regulator 1 Three Phase Ganged SVR : Subsystem
  Regulator 2 : Subsystem
  Regulator 3 : Subsystem
  Regulator 4 : Subsystem
  Regulator Taps : Subsystem
  Substation Power : Subsystem
  Three-Phase Transformer (Two Windings)1 : powerlib/Elements/Three-Phase Transformer (Two Windings)  Winding1Connection=Delta (D1)  Winding2Connection=Delta (D1)  CoreType=Three-limb core (core-type)  SetSaturation=off  Hysteresis=off  DataFile='hysteresis'  SetInitialFlux=off  Measurements=None  UNITS=pu  NominalPower=[150e3 ,60 ]  Winding1=[4160 0.0127 0.0272]  Winding2=[480 0.0127 0.0272]  Rm=1000  Lm=1000  L0=0.5  Saturation=[ 0,0 ; 0.0024,1.2 ; 1.0,1.52 ]  InitialFluxes=[ 0.8 , -0.8 , 0.7 ]  BreakLoop=on  DiscreteSolver=Trapezoidal iterative  DataType=off  TransfoNumber=1
      settings: SourceProductName=Simscape Electrical
  Three-Phase Breaker1 : powerlib/Elements/Three-Phase Breaker  InitialState=open  SwitchA=off  SwitchB=off  SwitchC=off  SwitchTimes="[1/60  5/60]"  External=off  BreakerResistance=0.01  SnubberResistance=1e6  SnubberCapacitance=inf  Measurements=None
      settings: SourceProductName=Simscape Electrical
  XF1 : powerlib/Measurements/Three-Phase V-I Measurement  VoltageMeasurement=phase-to-ground  SetLabelV=on  LabelV=XF1  Vpu=off  VpuLL=off  CurrentMeasurement=no  SetLabelI=on  LabelI=I65  Ipu=off  Pbase=100e6  Vbase=24900  OutputType=Complex  PhasorSimulation=on  PSBequivalent=0
      settings: SourceProductName=Simscape Electrical
  powergui : powerlib/powergui  Priority=1  SimulationMode=Phasor  SampleTime=Ts  frequency=60  Iterations=50  frequencyindice=0  Pbase=100e6  ErrMax=1e-4  UnitsV=kV  UnitsW=MW  buscounter=0  FunctionMessages=off  echomessages=on  EnableUseOfTLC=off  CurrentSourceSwitches=off  DisableSnubberDevices=off  DisableRonSwitches=off  DisableVfSwitches=off  DisplayEquations=off  AutomaticDiscreteSolvers=off  SolverType=Tustin/Backward Euler (TBE)  Interpol=off  ExternalGateDelay=off  methode=off  Ts=0  x0status=blocks  SPID=off  SwTol=0  HookPort=off  NonlinearTolerance=1e-4  nMaxIteration=100  ContinueOnMaxIteration=off  RestoreLinks=warning  ResistiveCurrentMeasurement=off  Frange=[0:2:500]  Ylog=off  Xlog=on  ShowGrid=off  save=off  variable=ZData  structure=0  ZoomFFT=off  StartTime=0.0  cycles=1  DisplayStyle=1  fundamental=60  FreqAxis=off  MaxFrequency=1000  frequencyindicesteady=1  RmsSteady=1  display=off
      settings: SourceProductName=Simscape Electrical
  tag scope: Reg1=global, Reg2=global, Reg3=global, Reg4=global
  wires:
  Regulator 1 Three Phase Ganged SVR/1(Tap) -> [Reg1]
  Regulator 4/1(Tap) -> [Reg4]
  Regulator 2/1(Tap) -> [Reg2]
  Regulator 3/1(Taps) -> [Reg3]
  connections:
  25-26 1/RConn1 -- 26-31 1/LConn1 -- 26/LConn2
  51-151 4/RConn3 -- 151/RConn3
  51-151 4/RConn2 -- 151/RConn2
  51-151 4/RConn1 -- 151/RConn1
  Regulator 1 Three Phase Ganged SVR/RConn3 -- RG1out/LConn3
  Regulator 1 Three Phase Ganged SVR/RConn2 -- RG1out/LConn2
  Regulator 1 Three Phase Ganged SVR/RConn1 -- RG1out/LConn1
  Regulator 1 Three Phase Ganged SVR/LConn3 -- RG1in/RConn3
  Regulator 1 Three Phase Ganged SVR/LConn2 -- RG1in/RConn2
  Regulator 1 Three Phase Ganged SVR/LConn1 -- RG1in/RConn1
  150/LConn2 -- 4160 V swing/RConn2
  4160 V swing/RConn3 -- 150/LConn3
  4160 V swing/RConn1 -- 150/LConn1
  Load Flow Bus2/LConn3 -- 35/RConn3
  Load Flow Bus2/LConn2 -- 35/RConn2
  Load Flow Bus2/LConn1 -- 35/RConn1
  Three-Phase Transformer (Two Windings)1/LConn3 -- XF1/RConn3
  RG1out/RConn3 -- 149/LConn3
  RG1out/RConn2 -- 149/LConn2
  RG1out/RConn1 -- 149/LConn1
  RG2out/RConn1 -- 14/LConn1
  160 67 6/RConn3 -- RG4in/LConn3
  160 67 6/RConn2 -- RG4in/LConn2
  160 67 6/RConn1 -- RG4in/LConn1
  9-14 9/RConn1 -- RG2in/LConn1
  610/RConn3 -- Load Flow Bus84/LConn3
  610/RConn2 -- Load Flow Bus84/LConn2
  610/RConn1 -- Load Flow Bus84/LConn1
  Three-Phase Transformer (Two Windings)1/RConn3 -- 610/LConn3
  Three-Phase Transformer (Two Windings)1/RConn2 -- 610/LConn2
  Three-Phase Transformer (Two Windings)1/RConn1 -- 610/LConn1
  Three-Phase Transformer (Two Windings)1/LConn2 -- XF1/RConn2
  Three-Phase Transformer (Two Windings)1/LConn1 -- XF1/RConn1
  85 Y PQ/LConn1 -- 85/RConn1
  75 Y PQ/LConn1 -- 75/RConn1
  71 Y PQ/LConn1 -- 71/RConn1
  103-104 11/RConn1 -- 104/LConn1
  106-107 10/RConn1 -- 107/LConn1
  114 Y PQ/LConn1 -- 114/RConn1
  111 Y PQ/LConn1 -- 111/RConn1
  87-88 9/RConn1 -- 88/LConn1
  89-90 10/RConn1 -- 90/LConn1
  91-92 11/RConn1 -- 92/LConn1
  96 Y PQ/LConn1 -- 96/RConn1
  15-17 11/RConn1 -- 17/LConn1
  15-16 11/RConn1 -- 16/LConn1
  59 Y PQ/LConn1 -- 59/RConn1
  57-58 10/LConn1 -- 58/LConn1
  36/RConn2 -- Load Flow Bus55/LConn2
  36/LConn2 -- 35-36 8/RConn2
  36/RConn1 -- Load Flow Bus55/LConn1
  37 Y Z/LConn1 -- 37/RConn1
  38-39 10/RConn1 -- 39/LConn1
  41 Y PQ/LConn1 -- 41/RConn1
  43 Y Z/LConn1 -- 43/RConn1
  45-46 9/RConn1 -- 46/LConn1
  31-32 1/RConn1 -- 32/LConn1
  33 Y I/LConn1 -- 33/RConn1
  27-33 1/LConn1 -- 27/RConn1
  23-24 11/RConn1 -- 24/LConn1
  21-22 10/RConn1 -- 22/LConn1
  20 Y I/LConn1 -- 20/RConn1
  95/RConn3 -- Load Flow Bus77/RConn3
  95/RConn2 -- Load Flow Bus77/RConn2
  95/RConn1 -- Load Flow Bus77/RConn1
  79/RConn3 -- Load Flow Bus117/LConn3
  79/RConn2 -- Load Flow Bus117/LConn2
  78-79 6/RConn3 -- 79/LConn3
  78-79 6/RConn2 -- 79/LConn2
  78-79 6/RConn1 -- 79/LConn1
  151/LConn3 -- 151-1/LConn3
  151/LConn2 -- 151-1/LConn2
  151/LConn1 -- 151-1/LConn1
  300/RConn3 -- Load Flow Bus44/LConn3
  300/RConn2 -- Load Flow Bus44/LConn2
  300/RConn1 -- Load Flow Bus44/LConn1
  450/RConn3 -- Load Flow Bus106/LConn3
  450/RConn2 -- Load Flow Bus106/LConn2
  450/RConn1 -- Load Flow Bus106/LConn1
  100-450 3/RConn3 -- 450/LConn3
  100-450 3/RConn2 -- 450/LConn2
  100-450 3/RConn1 -- 450/LConn1
  56/RConn3 -- Load Flow Bus68/LConn3
  56/RConn1 -- Load Flow Bus68/LConn1
  55-56 1/RConn3 -- 56/LConn3
  55-56 1/RConn2 -- 56/LConn2
  55-56 1/RConn1 -- 56/LConn1
  66/RConn2 -- Load Flow Bus128/LConn2
  66/RConn1 -- Load Flow Bus128/LConn1
  65-66 12/RConn3 -- 66/LConn3
  65-66 12/RConn2 -- 66/LConn2
  65-66 12/RConn1 -- 66/LConn1
  51-151 4/LConn3 -- 51/RConn3
  51-151 4/LConn2 -- 51/RConn2
  50-51 4/RConn3 -- 51/LConn3
  50-51 4/RConn2 -- 51/LConn2
  50-51 4/RConn1 -- 51/LConn1
  48 Y Z/LConn3 -- 48/LConn3
  48 Y Z/LConn2 -- 48/LConn2
  48 Y Z/LConn1 -- 48/LConn1
  8-12 10/RConn1 -- 12/LConn1
  6 Y Z/LConn1 -- 6/RConn1
  4Y PQ/LConn1 -- 4/RConn1
  11 Y Z/LConn1 -- 11/RConn1
  14-10 9/LConn1 -- 10/LConn1
  1-2 10/RConn1 -- 2/LConn1
  RG1in/LConn3 -- 150-1/RConn3
  RG1in/LConn2 -- 150-1/RConn2
  RG1in/LConn1 -- 150-1/RConn1
  1/RConn3 -- 1-3 11/LConn1 -- 1-7 1/LConn3
  1-7 1/LConn2 -- 1/RConn2
  1-7 1/LConn1 -- 1 Y PQ/LConn1 -- 1/RConn1
  Load Flow Bus44/RConn2 -- 300-1/LConn2
  Load Flow Bus44/RConn1 -- 300-1/LConn1
  300-1/RConn3 -- Load Flow Bus45/LConn3
  300-1/RConn2 -- Load Flow Bus45/LConn2
  300-1/RConn1 -- Load Flow Bus45/LConn1
  197/LConn3 -- 97-1/RConn3
  197/LConn2 -- 97-1/RConn2
  197/LConn1 -- 97-1/RConn1
  18-135/LConn3 -- 18-21 2/LConn3 -- 18/RConn3
  18-135/LConn2 -- 18-21 2/LConn2 -- 18/RConn2
  18-21 2/LConn1 -- 18-19 9/LConn1 -- 18-135/LConn1 -- 18/RConn1
  150/RConn3 -- 150-1/LConn3
  150/RConn1 -- 150-1/LConn1
  160 67 6/LConn1 -- 160/RConn1
  160 67 6/LConn2 -- 160/RConn2
  54/LConn1 -- 54-57 3/LConn1 -- 53-54 1/RConn1 -- 59-94/LConn1
  Three-Phase Breaker1/LConn3 -- 93-95 6/RConn3 -- 95/LConn3
  Three-Phase Breaker1/LConn2 -- 93-95 6/RConn2 -- 95 Y PQ/LConn1 -- 95/LConn2
  Three-Phase Breaker1/LConn1 -- 93-95 6/RConn1 -- 95/LConn1
  450-451/LConn3 -- Load Flow Bus106/RConn3
  Load Flow Bus106/RConn2 -- 450-451/LConn2
  Load Flow Bus106/RConn1 -- 450-451/LConn1
  Load Flow Bus44/RConn3 -- 300-1/LConn3
  250/RConn3 -- 250-251/LConn3
  250/RConn2 -- 250-251/LConn2
  250/RConn1 -- 250-251/LConn1
  135/LConn3 -- 18-135/RConn3
  135/LConn2 -- 18-135/RConn2
  135/LConn1 -- 18-135/RConn1
  35-40 1/RConn2 -- 40/LConn2
  35-40 1/RConn1 -- 40/LConn1
  35-40 1/RConn3 -- 40/LConn3
  77-78 6/LConn3 -- 77/RConn3
  77-78 6/LConn1 -- 77/RConn1
  77-78 6/LConn2 -- 77/RConn2
  87-89 6/LConn3 -- 87/RConn3
  87-89 6/LConn2 -- 87 Y PQ/LConn1 -- 87/RConn2
  34-15 11/RConn1 -- 15/LConn1
  64-65 12/LConn3 -- 64/RConn3
  64-65 12/LConn2 -- 64/RConn2
  64-65 12/LConn1 -- 64/RConn1
  110-112 9/LConn1 -- 110/RConn1
  54-55 1/RConn3 -- 55/LConn3
  54-55 1/RConn1 -- 55/LConn1
  54-55 1/RConn2 -- 55/LConn2
  73-74 11/RConn1 -- 74 Y Z/LConn1 -- 74/LConn1
  50-51 4/LConn3 -- 50/RConn3
  50-51 4/LConn2 -- 50/RConn2
  50-51 4/LConn1 -- 50/RConn1
  30-250 2/LConn3 -- "30 "/RConn3
  30-250 2/LConn2 -- "30 "/RConn2
  30-250 2/LConn1 -- "30 "/RConn1
  98-99 3/LConn3 -- 98/RConn3
  98-99 3/LConn2 -- 98/RConn2
  98-99 3/LConn1 -- 98 Y PQ/LConn1 -- 98/RConn1
  57-60 3/LConn1 -- 57/LConn1
  57-60 3/LConn3 -- 57/LConn3
  57-60 3/LConn2 -- 57/LConn2
  7-8 1/LConn3 -- 7/RConn3
  7-8 1/LConn2 -- 7/RConn2
  7-8 1/LConn1 -- 7/RConn1
  91-93 6/RConn1 -- 93/LConn1
  91-93 6/RConn3 -- 93/LConn3
  91-93 6/RConn2 -- 93/LConn2
  81-82 6/LConn2 -- 81/RConn2
  81-82 6/LConn1 -- 81/RConn1
  72-76 3/LConn3 -- 72/RConn3
  72-76 3/LConn2 -- 72/RConn2
  72-76 3/LConn1 -- 72/RConn1
  101-105 3/LConn3 -- 101/RConn3
  101-105 3/LConn2 -- 101/RConn2
  101-105 3/LConn1 -- 101/RConn1
  108-300 3/LConn3 -- 108/RConn3
  108-300 3/LConn2 -- 108/RConn2
  108/RConn1 -- 108-300 3/LConn1 -- 108-109 9/LConn1
  44-47 1/LConn3 -- 44/RConn3
  44-47 1/LConn2 -- 44/RConn2
  25-28 2/LConn3 -- 25/RConn3
  25-28 2/LConn2 -- 25/RConn2
  25-28 2/LConn1 -- 25/RConn1
  160 67 6/LConn3 -- 160/RConn3
  13-152/RConn3 -- 152/LConn3
  13-152/RConn2 -- 152/LConn2
  13-152/RConn1 -- 152/LConn1
  64-65 12/RConn1 -- 65 D Z/LConn1 -- 65/LConn1
  64-65 12/RConn3 -- 65 D Z/LConn3 -- 65/LConn3
  55-56 1/LConn1 -- 55 Y Z/LConn1 -- 55/RConn1
  55-56 1/LConn2 -- 55/RConn2
  55-56 1/LConn3 -- 55/RConn3
  51-151 4/LConn1 -- 51 Y PQ/LConn1 -- 51/RConn1
  21-23 2/LConn1 -- 21/RConn1
  27-33 1/RConn1 -- 33/LConn1
  67-72 3/RConn3 -- 72/LConn3
  Load Flow Bus68/LConn2 -- 56 Y PQ/LConn1 -- 56/RConn2
  25/LConn3 -- 23-25 2/RConn3 -- RG3in/LConn2
  74-75 11/RConn1 -- 75/LConn1
  47-48 4/RConn2 -- 47 Y I/LConn2 -- 47/LConn2
  73/LConn1 -- 73 Y PQ/LConn1 -- 72-73 11/RConn1
  70-71 1/RConn1 -- 71/LConn1
  28-29 2/RConn3 -- 29/LConn3
  70-71 1/LConn1 -- 70 Y PQ/LConn1 -- 70/RConn1
  17 Y PQ/LConn1 -- 17/RConn1
  21/RConn2 -- 21-23 2/LConn2 -- 21-22 10/LConn1
  69-70 9/RConn1 -- 70/LConn1
  54-55 1/LConn3 -- 54/RConn3
  35/LConn1 -- 135-35 4/RConn1 -- 35-40 1/LConn1
  60/LConn2 -- 60-62 12/LConn2 -- 60-61 5/LConn2 -- 60-1/LConn2
  12 Y PQ/LConn1 -- 12/RConn1
  1-7 1/RConn2 -- 7/LConn2
  67-72 3/LConn2 -- 67/LConn2
  87-89 6/RConn2 -- 89/LConn2
  86-87 6/RConn2 -- 87/LConn2
  8-13 1/LConn3 -- 8/RConn3
  8-13 1/RConn1 -- 13/LConn1
  8-13 1/LConn2 -- 8/RConn2
  8/LConn1 -- 7-8 1/RConn1 -- 8-9 9/LConn1
  93-95 6/LConn2 -- 93/RConn2
  89/RConn2 -- 89-91 6/LConn2 -- 89-90 10/LConn1
  16 Y PQ/LConn1 -- 16/RConn1
  5/LConn1 -- 3-5 11/RConn1
  3-4 11/RConn1 -- 4/LConn1
  13/LConn3 -- 8-13 1/RConn3 -- 13-34 11/LConn1
  9/RConn1 -- 9-14 9/LConn1 -- 9 Y PQ/LConn1
  13/RConn1 -- 13-18 2/LConn1 -- 13-152/LConn1
  13/RConn3 -- 13-18 2/LConn3 -- 13-152/LConn3
  13-18 2/RConn2 -- 18/LConn2
  13-18 2/RConn1 -- 18/LConn1
  13-18 2/RConn3 -- 18/LConn3
  10 Y I/LConn1 -- 10/RConn1
  14/RConn1 -- 14-11 9/LConn1 -- 14-10 9/RConn1
  8-13 1/LConn1 -- 8/RConn1
  7/LConn1 -- 7 Y PQ/LConn1 -- 1-7 1/RConn1
  1-7 1/RConn3 -- 7/LConn3
  47-49 4/LConn1 -- 47/RConn1
  15/RConn1 -- 15-16 11/LConn1 -- 15-17 11/LConn1
  42-44 1/LConn1 -- 42/RConn1
  14-11 9/RConn1 -- 11/LConn1
  13-34 11/RConn1 -- 34/LConn1
  52-53 1/RConn3 -- 53/LConn3
  1-3 11/RConn1 -- 3/LConn1
  57/RConn2 -- 57-58 10/RConn1 -- 54-57 3/RConn2
  18-21 2/RConn3 -- 21/LConn3
  73-74 11/LConn1 -- 73/RConn1
  74-75 11/LConn1 -- 74/RConn1
  53-54 1/LConn1 -- 53/RConn1
  52-53 1/LConn2 -- 52/RConn2
  53-54 1/LConn3 -- 53/RConn3
  52-53 1/RConn2 -- 53/LConn2
  18-21 2/RConn2 -- 21/LConn2
  Load Flow Bus2/RConn1 -- 35 D PQ/LConn1 -- 35-36 8/LConn1
  52-53 1/RConn1 -- 53 Y PQ/LConn1 -- 53/LConn1
  52-53 1/LConn3 -- 52/RConn3
  53-54 1/LConn2 -- 53/RConn2
  35/LConn2 -- 135-35 4/RConn2 -- 35-40 1/LConn2
  65-66 12/LConn2 -- 65/RConn2
  62-63 12/RConn3 -- 63/LConn3
  58-59 10/RConn1 -- 58 Y I/LConn1 -- 58/RConn1
  6/LConn1 -- 5-6 11/RConn1
  19-20 9/LConn1 -- 19/RConn1
  57-60 3/RConn1 -- 60/RConn1
  5/RConn1 -- 5 Y I/LConn1 -- 5-6 11/LConn1
  63-64 12/LConn1 -- 63/RConn1
  63-64 12/LConn2 -- 63/RConn2
  69/RConn1 -- 69 Y PQ/LConn1 -- 69-70 9/LConn1
  60-62 12/RConn1 -- 62/LConn1
  24 Y PQ/LConn1 -- 24/RConn1
  28-29 2/RConn2 -- 29/LConn2
  54-57 3/RConn1 -- 57/RConn1
  29-30 2/LConn1 -- 29/RConn1
  60/LConn3 -- 60-62 12/LConn3 -- 60-61 5/LConn3 -- 60-1/LConn3
  2 Y PQ/LConn1 -- 2/RConn1
  97-98 3/RConn2 -- 98/LConn2
  63-64 12/LConn3 -- 63/RConn3
  8-13 1/RConn2 -- 13/LConn2
  8/LConn2 -- 7-8 1/RConn2 -- 8-12 10/LConn1
  42/RConn2 -- 42-43 10/LConn1 -- 42-44 1/LConn2
  3/RConn1 -- 3-4 11/LConn1 -- 3-5 11/LConn1
  1/LConn2 -- 1-2 10/LConn1 -- 149-1 1/RConn2
  13/RConn2 -- 13-18 2/LConn2 -- 13-152/LConn2
  8-9 9/RConn1 -- 9/LConn1
  7-8 1/RConn3 -- 8/LConn3
  76/LConn1 -- 76-77 6/LConn1 -- 72-76 3/RConn1
  52-53 1/LConn1 -- 52/RConn1
  40/RConn3 -- 40-41 11/LConn1 -- 40-42 1/LConn3
  28-29 2/LConn3 -- 28/RConn3
  38-39 10/LConn1 -- 38 Y I/LConn1 -- 38/RConn1
  54-57 3/RConn3 -- 57/RConn3
  40-41 11/RConn1 -- 41/LConn1
  57-60 3/RConn2 -- 60/RConn2
  60/LConn1 -- 60 Y PQ/LConn1 -- 60-62 12/LConn1 -- 60-61 5/LConn1 -- 60-1/LConn1
  18-21 2/RConn1 -- 21/LConn1
  23/RConn3 -- 23-25 2/LConn3 -- 23-24 11/LConn1
  29-30 2/LConn2 -- 29/RConn2
  29-30 2/RConn1 -- "30 "/LConn1
  44/RConn1 -- 44-45 9/LConn1 -- 44-47 1/LConn1
  60-62 12/RConn2 -- 62/LConn2
  63-64 12/RConn1 -- 64/LConn1
  67-97 3/RConn2 -- 97/LConn2
  29-30 2/LConn3 -- 29/RConn3
  67/RConn2 -- 67-97 3/LConn2 -- RG4out/RConn2
  29/LConn1 -- 29 Y Z/LConn1 -- 28-29 2/RConn1
  47-48 4/RConn3 -- 47 Y I/LConn3 -- 47/LConn3
  76/LConn2 -- 76-77 6/LConn2 -- 72-76 3/RConn2
  76/LConn3 -- 76-77 6/LConn3 -- 72-76 3/RConn3
  57-60 3/RConn3 -- 60/RConn3
  28-29 2/LConn1 -- 28/RConn1
  28-29 2/LConn2 -- 28/RConn2
  62-63 12/RConn2 -- 63/LConn2
  54/LConn3 -- 54-57 3/LConn3 -- 53-54 1/RConn3
  22 Y Z/LConn1 -- 22/RConn1
  49-50 4/LConn3 -- 49/RConn3
  21-23 2/RConn2 -- 23/LConn2
  67-97 3/LConn1 -- RG4out/RConn1 -- 67-68 9/LConn1 -- 67/RConn1
  62-63 12/LConn3 -- 62/RConn3
  45-46 9/LConn1 -- 45/RConn1
  47-49 4/RConn1 -- 49 Y PQ/LConn1 -- 49/LConn1
  29-30 2/RConn3 -- 30 Y PQ/LConn1 -- "30 "/LConn3
  54-55 1/LConn1 -- 54/RConn1
  21-23 2/RConn3 -- 23/LConn3
  30-250 2/RConn1 -- 250/LConn1
  26-31 1/RConn1 -- 31/LConn1
  40-42 1/LConn1 -- 40/RConn1
  23-25 2/LConn2 -- 23/RConn2
  65-66 12/LConn3 -- 65/RConn3
  Load Flow Bus128/LConn3 -- 66 Y PQ/LConn1 -- 66/RConn3
  67-72 3/LConn1 -- 67/LConn1
  68-69 9/RConn1 -- 69/LConn1
  29-30 2/RConn2 -- "30 "/LConn2
  60-62 12/RConn3 -- 62 Y Z/LConn1 -- 62/LConn3
  21-23 2/RConn1 -- 23/LConn1
  18-19 9/RConn1 -- 19 Y PQ/LConn1 -- 19/LConn1
  58-59 10/LConn1 -- 59/LConn1
  67-72 3/RConn1 -- 72/LConn1
  23-25 2/RConn2 -- 25/LConn2
  48/RConn2 -- 44-47 1/RConn2 -- 47-48 4/LConn2
  67-68 9/RConn1 -- 68/LConn1
  49-50 4/LConn1 -- 49/RConn1
  65-66 12/LConn1 -- 65/RConn1
  48/RConn1 -- 44-47 1/RConn1 -- 47-48 4/LConn1
  62-63 12/RConn1 -- 63 Y PQ/LConn1 -- 63/LConn1
  25-28 2/RConn3 -- 28/LConn3
  21-23 2/LConn3 -- 21/RConn3
  62-63 12/LConn2 -- 62/RConn2
  46 Y PQ/LConn1 -- 46/RConn1
  47-48 4/RConn1 -- 47 Y I/LConn1 -- 47/LConn1
  67/LConn3 -- 67-72 3/LConn3 -- 72-73 11/LConn1
  62-63 12/LConn1 -- 62/RConn1
  63-64 12/RConn2 -- 64 Y I/LConn1 -- 64/LConn2
  48/RConn3 -- 44-47 1/RConn3 -- 47-48 4/LConn3
  25-28 2/RConn2 -- 28/LConn2
  25-28 2/RConn1 -- 28 Y I/LConn1 -- 28/LConn1
  31-32 1/LConn1 -- 31/RConn1 -- 31 Y PQ/LConn1
  30-250 2/RConn2 -- 250/LConn2
  34/RConn1 -- 34 Y Z/LConn1 -- 34-15 11/LConn1
  35/LConn3 -- 135-35 4/RConn3 -- 35-40 1/LConn3
  36-37 9/RConn1 -- 37/LConn1
  36-38 10/LConn1 -- Load Flow Bus55/RConn2
  36-38 10/RConn1 -- 38/LConn1
  67-97 3/RConn1 -- 97/LConn1
  30-250 2/RConn3 -- 250/LConn3
  32 Y PQ/LConn1 -- 32/RConn1
  49-50 4/RConn1 -- 50/LConn1
  40-42 1/RConn3 -- 42/LConn3
  40-42 1/RConn2 -- 42/LConn2
  42-44 1/RConn3 -- 44/LConn3
  42-44 1/RConn2 -- 44/LConn2
  68-69 9/LConn1 -- 68 Y PQ/LConn1 -- 68/RConn1
  42-44 1/RConn1 -- 44/LConn1
  42-43 10/RConn1 -- 43/LConn1
  40-42 1/RConn1 -- 42 Y PQ/LConn1 -- 42/LConn1
  47-49 4/LConn3 -- 47/RConn3
  42-44 1/LConn3 -- 42/RConn3
  39 Y PQ/LConn1 -- 39/RConn1
  64-65 12/RConn2 -- 65 D Z/LConn2 -- 65/LConn2
  40-42 1/LConn2 -- 40/RConn2
  49-50 4/RConn2 -- 50/LConn2
  49-50 4/RConn3 -- 50 Y PQ/LConn1 -- 50/LConn3
  67-97 3/RConn3 -- 97/LConn3
  45/LConn1 -- 45 Y I/LConn1 -- 44-45 9/RConn1
  23-25 2/LConn1 -- 23/RConn1
  67/RConn3 -- 67-97 3/LConn3 -- RG4out/RConn3
  19-20 9/RConn1 -- 20/LConn1
  35-36 8/LConn2 -- 35 D PQ/RConn1 -- Load Flow Bus2/RConn2
  67-72 3/RConn2 -- 72/LConn2
  54-55 1/LConn2 -- 54/RConn2
  25/LConn1 -- 23-25 2/RConn1 -- RG3in/LConn1
  47-49 4/RConn3 -- 49 Y PQ/LConn3 -- 49/LConn3
  47-49 4/RConn2 -- 49 Y PQ/LConn2 -- 49/LConn2
  49-50 4/LConn2 -- 49/RConn2
  47-49 4/LConn2 -- 47/RConn2
  63-64 12/RConn3 -- 64/LConn3
  36/LConn1 -- 36-37 9/LConn1 -- 35-36 8/RConn1
  54/LConn2 -- 54-57 3/LConn2 -- 53-54 1/RConn2
  10 Y I/RConn1 -- Ground7/LConn1
  250-251/RConn2 -- Load Flow Bus10/LConn2
  7 Y PQ/RConn1 -- Ground5/LConn1
  5 Y I/RConn1 -- Ground4/LConn1
  2 Y PQ/RConn1 -- Ground1/LConn1
  76-86 3/RConn1 -- 86/LConn1
  60-61 5/RConn3 -- 61/LConn3
  9 Y PQ/RConn1 -- Ground6/LConn1
  94/LConn1 -- 59-94/RConn1
  450-451/RConn2 -- Load Flow Bus107/LConn2
  11 Y Z/RConn1 -- Ground8/LConn1
  6 Y Z/RConn1 -- Ground3/LConn1
  77-78 6/RConn2 -- 78/LConn2
  77-78 6/RConn1 -- 78/LConn1
  Load Flow Bus78/LConn1 -- Three-Phase Breaker1/RConn1
  76-86 3/LConn3 -- 76 DI/LConn3 -- 76/RConn3
  76-86 3/RConn2 -- 86/LConn2
  60-61 5/RConn2 -- 61/LConn2
  Load Flow Bus78/LConn3 -- Three-Phase Breaker1/RConn3
  1 Y PQ/RConn1 -- Ground/LConn1
  Load Flow Bus78/LConn2 -- Three-Phase Breaker1/RConn2
  12 Y PQ/RConn1 -- Ground9/LConn1
  16 Y PQ/RConn1 -- Ground10/LConn1
  17 Y PQ/RConn1 -- Ground11/LConn1
  19 Y PQ/RConn1 -- Ground12/LConn1
  20 Y I/RConn1 -- Ground13/LConn1
  22 Y Z/RConn1 -- Ground14/LConn1
  24 Y PQ/RConn1 -- Ground15/LConn1
  28 Y I/RConn1 -- Ground16/LConn1
  29 Y Z/RConn1 -- Ground17/LConn1
  30 Y PQ/RConn1 -- Ground18/LConn1
  31 Y PQ/RConn1 -- Ground19/LConn1
  32 Y PQ/RConn1 -- Ground20/LConn1
  33 Y I/RConn1 -- Ground21/LConn1
  34 Y Z/RConn1 -- Ground22/LConn1
  37 Y Z/RConn1 -- Ground23/LConn1
  38 Y I/RConn1 -- Ground24/LConn1
  39 Y PQ/RConn1 -- Ground25/LConn1
  41 Y PQ/RConn1 -- Ground26/LConn1
  42 Y PQ/RConn1 -- Ground27/LConn1
  43 Y Z/RConn1 -- Ground28/LConn1
  45 Y I/RConn1 -- Ground29/LConn1
  46 Y PQ/RConn1 -- Ground30/LConn1
  50 Y PQ/RConn1 -- Ground31/LConn1
  51 Y PQ/RConn1 -- Ground32/LConn1
  52 Y PQ/RConn1 -- Ground33/LConn1
  53 Y PQ/RConn1 -- Ground34/LConn1
  55 Y Z/RConn1 -- Ground35/LConn1
  56 Y PQ/RConn1 -- Ground36/LConn1
  58 Y I/RConn1 -- Ground37/LConn1
  59 Y PQ/RConn1 -- Ground38/LConn1
  60 Y PQ/RConn1 -- Ground39/LConn1
  62 Y Z/RConn1 -- Ground40/LConn1
  63 Y PQ/RConn1 -- Ground41/LConn1
  64 Y I/RConn1 -- Ground42/LConn1
  66 Y PQ/RConn1 -- Ground43/LConn1
  68 Y PQ/RConn1 -- Ground44/LConn1
  69 Y PQ/RConn1 -- Ground45/LConn1
  70 Y PQ/RConn1 -- Ground46/LConn1
  71 Y PQ/RConn1 -- Ground47/LConn1
  73 Y PQ/RConn1 -- Ground48/LConn1
  74 Y Z/RConn1 -- Ground49/LConn1
  75 Y PQ/RConn1 -- Ground50/LConn1
  77 Y PQ/RConn1 -- Ground51/LConn1
  79 Y Z/RConn1 -- Ground52/LConn1
  80 Y PQ/RConn1 -- Ground53/LConn1
  82 Y PQ/RConn1 -- Ground54/LConn1
  83 Y PQ/RConn1 -- Ground55/LConn1
  84 Y PQ/RConn1 -- Ground56/LConn1
  85 Y PQ/RConn1 -- Ground57/LConn1
  86 Y PQ/RConn1 -- Ground58/LConn1
  87 Y PQ/RConn1 -- Ground59/LConn1
  88 Y PQ/RConn1 -- Ground60/LConn1
  90 Y I/RConn1 -- Ground61/LConn1
  92 Y PQ/RConn1 -- Ground62/LConn1
  94 Y PQ/RConn1 -- Ground63/LConn1
  95 Y PQ/RConn1 -- Ground64/LConn1
  96 Y PQ/RConn1 -- Ground65/LConn1
  98 Y PQ/RConn1 -- Ground66/LConn1
  99 Y PQ/RConn1 -- Ground67/LConn1
  100 Y Z/RConn1 -- Ground68/LConn1
  102 Y PQ/RConn1 -- Ground69/LConn1
  103 Y PQ/RConn1 -- Ground70/LConn1
  104 Y PQ/RConn1 -- Ground71/LConn1
  106 Y PQ/RConn1 -- Ground72/LConn1
  107 Y PQ/RConn1 -- Ground73/LConn1
  109 Y PQ/RConn1 -- Ground74/LConn1
  111 Y PQ/RConn1 -- Ground75/LConn1
  112 Y I/RConn1 -- Ground76/LConn1
  113 Y Z/RConn1 -- Ground77/LConn1
  114 Y PQ/RConn1 -- Ground78/LConn1
  83/RConn1 -- 83 Y CAP/LConn1
  83/RConn2 -- 83 Y CAP/LConn2
  83/RConn3 -- 83 Y CAP/LConn3
  Ground79/LConn1 -- 88 Y CAP/RConn1
  Ground80/LConn1 -- 90 Y CAP/RConn1
  Ground81/LConn1 -- 92 Y CAP/RConn1
  149-1 1/RConn3 -- 1/LConn3
  149-1 1/LConn3 -- 149/RConn3
  197-101 3/RConn2 -- 101/LConn2
  76-86 3/LConn2 -- 76 DI/LConn2 -- 76/RConn2
  77-78 6/RConn3 -- 78/LConn3
  100-450 3/LConn1 -- 100/RConn1
  78/RConn1 -- 78-80 6/LConn1 -- 78-79 6/LConn1
  99-100 3/RConn1 -- 100/LConn1
  78/RConn3 -- 78-80 6/LConn3 -- 78-79 6/LConn3
  99-100 3/RConn2 -- 100/LConn2
  99-100 3/RConn3 -- 100/LConn3
  99-100 3/LConn2 -- 99 Y PQ/LConn1 -- 99/RConn2
  76-77 6/RConn3 -- 77/LConn3
  77/LConn2 -- 77 Y PQ/LConn1 -- 76-77 6/RConn2
  76-77 6/RConn1 -- 77/LConn1
  149-1 1/LConn2 -- 149/RConn2
  149-1 1/RConn1 -- 1/LConn1
  197-101 3/RConn3 -- 101/LConn3
  149-1 1/LConn1 -- 149/RConn1
  135-35 4/LConn3 -- 135/RConn3
  152-52 1/RConn1 -- 52 Y PQ/LConn1 -- 52/LConn1
  135-35 4/LConn2 -- 135/RConn2
  135-35 4/LConn1 -- 135/RConn1
  152-52 1/RConn2 -- 52/LConn2
  113-114 9/RConn1 -- 114/LConn1
  113-114 9/LConn1 -- 113 Y Z/LConn1 -- 113/RConn1
  152-52 1/RConn3 -- 52/LConn3
  112-113 9/RConn1 -- 113/LConn1
  152-52 1/LConn1 -- 152/RConn1
  112/RConn1 -- 112 Y I/LConn1 -- 112-113 9/LConn1
  110-112 9/RConn1 -- 112/LConn1
  152-52 1/LConn2 -- 152/RConn2
  110-111 9/RConn1 -- 111/LConn1
  152-52 1/LConn3 -- 152/RConn3
  110/LConn1 -- 110-111 9/LConn1 -- 109-110 9/RConn1
  109/RConn1 -- 109 Y PQ/LConn1 -- 109-110 9/LConn1
  450-451/RConn3 -- Load Flow Bus107/LConn3
  250-251/RConn3 -- Load Flow Bus10/LConn3
  300/LConn3 -- 108-300 3/RConn3 -- 151-1/RConn3
  300/LConn2 -- 108-300 3/RConn2 -- 151-1/RConn2
  300/LConn1 -- 108-300 3/RConn1 -- 151-1/RConn1
  108-109 9/RConn1 -- 109/LConn1
  107 Y PQ/LConn1 -- 107/RConn1
  106-107 10/LConn1 -- 106 Y PQ/LConn1 -- 106/RConn1
  60-61 5/RConn1 -- 61/LConn1
  105/RConn2 -- 105-108 3/LConn2 -- 105-106 10/LConn1
  105-108 3/LConn3 -- 105/RConn3
  105-108 3/LConn1 -- 105/RConn1
  105-108 3/RConn3 -- 108/LConn3
  105-108 3/RConn2 -- 108/LConn2
  105-108 3/RConn1 -- 108/LConn1
  105-106 10/RConn1 -- 106/LConn1
  60-1/RConn1 -- 160/LConn1
  101-105 3/RConn2 -- 105/LConn2
  60-1/RConn2 -- 160/LConn2
  105/LConn3 -- 101-102 11/LConn1 -- 101-105 3/RConn3
  60-1/RConn3 -- 160/LConn3
  101-105 3/RConn1 -- 105/LConn1
  103-104 11/LConn1 -- 103 Y PQ/LConn1 -- 103/RConn1
  104 Y PQ/LConn1 -- 104/RConn1
  197-101 3/LConn2 -- 197/RConn2
  102-103 11/RConn1 -- 103/LConn1
  102/RConn1 -- 102 Y PQ/LConn1 -- 102-103 11/LConn1
  197-101 3/LConn3 -- 197/RConn3
  101-102 11/RConn1 -- 102/LConn1
  197-101 3/RConn1 -- 101/LConn1
  100-450 3/LConn3 -- 100 Y Z/LConn1 -- 100/RConn3
  100-450 3/LConn2 -- 100/RConn2
  92/RConn1 -- 92 Y PQ/LConn1 -- 92 Y CAP/LConn1
  91/RConn3 -- 91-93 6/LConn3 -- 91-92 11/LConn1
  4Y PQ/RConn1 -- Ground2/LConn1
  89-91 6/RConn3 -- 91/LConn3
  89-91 6/RConn2 -- 91/LConn2
  89-91 6/RConn1 -- 91/LConn1
  93/RConn1 -- 93-95 6/LConn1 -- 93-94 9/LConn1
  89-91 6/LConn3 -- 89/RConn3
  89-91 6/LConn1 -- 89/RConn1
  90 Y CAP/LConn1 -- 90 Y I/LConn1 -- 90/RConn1
  87-89 6/RConn3 -- 89/LConn3
  87-89 6/RConn1 -- 89/LConn1
  87/RConn1 -- 87-89 6/LConn1 -- 87-88 9/LConn1
  450-451/RConn1 -- Load Flow Bus107/LConn1
  88 Y CAP/LConn1 -- 88 Y PQ/LConn1 -- 88/RConn1
  95-96 10/LConn1 -- Load Flow Bus77/LConn2
  86-87 6/RConn3 -- 87/LConn3
  86-87 6/RConn1 -- 87/LConn1
  93-95 6/LConn3 -- 93/RConn3
  86-87 6/LConn3 -- 86/RConn3
  86-87 6/LConn2 -- 86 Y PQ/LConn1 -- 86/RConn2
  97-98 3/RConn1 -- 98/LConn1
  150/RConn2 -- 150-1/LConn2
  86-87 6/LConn1 -- 86/RConn1
  95-96 10/RConn1 -- 96/LConn1
  82-83 6/RConn3 -- 83 Y PQ/LConn1 -- 83/LConn3
  97-98 3/RConn3 -- 98/LConn3
  82-83 6/RConn2 -- 83/LConn2
  82-83 6/RConn1 -- 83/LConn1
  82-83 6/LConn3 -- 82/RConn3
  82-83 6/LConn2 -- 82/RConn2
  82-83 6/LConn1 -- 82 Y PQ/LConn1 -- 82/RConn1
  84-85 11/RConn1 -- 85/LConn1
  84-85 11/LConn1 -- 84/RConn1
  98-99 3/RConn1 -- 99/LConn1
  81-84 11/RConn1 -- 84 Y PQ/LConn1 -- 84/LConn1
  250-251/RConn1 -- Load Flow Bus10/LConn1
  98-99 3/RConn2 -- 99/LConn2
  81-82 6/RConn3 -- 82/LConn3
  81-82 6/RConn2 -- 82/LConn2
  98-99 3/RConn3 -- 99/LConn3
  81-82 6/RConn1 -- 82/LConn1
  81/RConn3 -- 81-84 11/LConn1 -- 81-82 6/LConn3
  99-100 3/LConn1 -- 99/RConn1
  76-86 3/LConn1 -- 76 DI/LConn1 -- 76/RConn1
  91-93 6/LConn1 -- 91/RConn1
  80-81 6/RConn3 -- 81/LConn3
  91-93 6/LConn2 -- 91/RConn2
  80-81 6/RConn2 -- 81/LConn2
  80-81 6/RConn1 -- 81/LConn1
  80-81 6/LConn3 -- 80/RConn3
  93-94 9/RConn1 -- 94 Y PQ/LConn1 -- 94/RConn1
  80-81 6/LConn2 -- 80 Y PQ/LConn1 -- 80/RConn2
  80-81 6/LConn1 -- 80/RConn1
  78-80 6/RConn3 -- 80/LConn3
  78-80 6/RConn2 -- 80/LConn2
  97-1/LConn1 -- 97-98 3/LConn1 -- 97/RConn1
  97/RConn3 -- 97-98 3/LConn3 -- 97-1/LConn3
  97-1/LConn2 -- 97-98 3/LConn2 -- 97/RConn2
  197-101 3/LConn1 -- 197/RConn1
  99-100 3/LConn3 -- 99/RConn3
  76-86 3/RConn3 -- 86/LConn3
  Load Flow Bus117/LConn1 -- 79 Y Z/LConn1 -- 79/RConn1
  78/RConn2 -- 78-80 6/LConn2 -- 78-79 6/LConn2
  78-80 6/RConn1 -- 80/LConn1
  Regulator 4/LConn1 -- RG4in/RConn1
  RG4in/RConn2 -- Regulator 4/LConn2
  RG4in/RConn3 -- Regulator 4/LConn3
  Regulator 4/RConn1 -- RG4out/LConn1
  Regulator 4/RConn2 -- RG4out/LConn2
  Regulator 4/RConn3 -- RG4out/LConn3
  Regulator 2/LConn1 -- RG2in/RConn1
  Regulator 2/RConn1 -- RG2out/LConn1
  26/RConn1 -- 26-27 7/LConn2
  26-27 7/RConn2 -- 27/LConn1
  27/LConn2 -- 26-27 7/RConn1
  26/RConn2 -- 26-27 7/LConn1
  26/LConn1 -- 25-26 1/RConn2
  25-26 1/LConn2 -- RG3out/RConn1
  25-26 1/LConn1 -- RG3out/RConn2
  Regulator 3/RConn1 -- RG3out/LConn1
  Regulator 3/RConn2 -- RG3out/LConn2
  Regulator 3/LConn1 -- RG3in/RConn1
  Regulator 3/LConn2 -- RG3in/RConn2
  61-610/LConn1 -- 61/RConn1
  61-610/LConn2 -- 61/RConn2
  61-610/LConn3 -- 61/RConn3
  61-610/RConn1 -- XF1/LConn1
  61-610/RConn2 -- XF1/LConn2
  61-610/RConn3 -- XF1/LConn3
